simulink model "v2012_PF"  (Simulink 7.6)
(part 2 of 4)

  Line133 : PMComponent  Tag=PSATblock  Description=Power Flow  PhysicalDomain=psatdomain  LeftPortType=p1  RightPortType=p1  LConnTagsString=__newl0  RConnTagsString=__newr0  mask(Line){p3_4_5q=[100  230  60], p6q=9, p8q=[0.023], p9q=[0.00036046], p10q=[0.357e-6], p13_14_15q=[475.8 432.5 475.8], p16q=on}
      mask prompts: p3_4_5q "Power, Voltage and Frequency Ratings [MVA, kV, Hz]"; p6q "Length of line [km] (0 for p.u. parameters)"; p8q "Resistance [p.u. (Ohms/km)]"; p9q "Reactance [p.u. (H/km)]"; p10q "Susceptance [p.u. (F/km)]"; p13_14_15q "Imax, Pmax and Smax [p.u., p.u., p.u.]"; p16q "Connected"
      mask help: This block defines a pi model for a tree phase cable.
      mask init:
      | [x,y] = fm_draw('circle');
      | [x1,y1] = fm_draw('semicircle');
      mask CallbackString: ||||||fm_block
      mask Display:
      | color('yellow')
      | plot(10+0.433*x,0.5+0.433*y)
      | plot(9.567+0.433*x,-0.25+0.433*y)
      | plot(10.433+0.433*x,-0.25+0.433*y)
      | color('black')
      | plot(-x1,y1)
      | plot(10+x,y,[0 10],[1 1],[0 10],[-1 -1])
  Line134 : PMComponent  Tag=PSATblock  Description=Power Flow  PhysicalDomain=psatdomain  LeftPortType=p1  RightPortType=p1  LConnTagsString=__newl0  RConnTagsString=__newr0  mask(Line){p3_4_5q=[100  230  60], p6q=19, p8q=[0.05], p9q=[0.001294461], p10q=[0.008941863e-6], p13_14_15q=[62.8 57.1 62.8], p16q=on}
      mask prompts: p3_4_5q "Power, Voltage and Frequency Ratings [MVA, kV, Hz]"; p6q "Length of line [km] (0 for p.u. parameters)"; p8q "Resistance [p.u. (Ohms/km)]"; p9q "Reactance [p.u. (H/km)]"; p10q "Susceptance [p.u. (F/km)]"; p13_14_15q "Imax, Pmax and Smax [p.u., p.u., p.u.]"; p16q "Connected"
      mask help: This block defines a pi model for a tree phase line.
      mask init:
      | [xp,yp] = fm_draw('pi');
      mask CallbackString: ||||||fm_block
      mask Display:
      | plot([-1  1  1 -1 -1],[-0.2 -0.2 0.2 0.2 -0.2])
      | color('blue')
      | plot(0.35*xp,0.2*yp)
  Line135 : PMComponent  Tag=PSATblock  Description=Power Flow  PhysicalDomain=psatdomain  LeftPortType=p1  RightPortType=p1  LConnTagsString=__newl0  RConnTagsString=__newr0  mask(Line){p3_4_5q=[100  138  60], p6q=15.4, p8q=[0.125], p9q=[0.000994719], p10q=[0.007460394e-6], p13_14_15q=[36.3 33 36.3], p16q=on}
      mask prompts: p3_4_5q "Power, Voltage and Frequency Ratings [MVA, kV, Hz]"; p6q "Length of line [km] (0 for p.u. parameters)"; p8q "Resistance [p.u. (Ohms/km)]"; p9q "Reactance [p.u. (H/km)]"; p10q "Susceptance [p.u. (F/km)]"; p13_14_15q "Imax, Pmax and Smax [p.u., p.u., p.u.]"; p16q "Connected"
      mask help: This block defines a pi model for a tree phase line.
      mask init:
      | [xp,yp] = fm_draw('pi');
      mask CallbackString: ||||||fm_block
      mask Display:
      | plot([-1  1  1 -1 -1],[-0.2 -0.2 0.2 0.2 -0.2])
      | color('blue')
      | plot(0.35*xp,0.2*yp)
  Line136 : PMComponent  Tag=PSATblock  Description=Power Flow  PhysicalDomain=psatdomain  LeftPortType=p1  RightPortType=p1  LConnTagsString=__newl0  RConnTagsString=__newr0  mask(Line){p3_4_5q=[100  138  60], p6q=15.4, p8q=[0.125], p9q=[0.000994719], p10q=[0.007460394e-6], p13_14_15q=[36.3 33 36.3], p16q=on}
      mask prompts: p3_4_5q "Power, Voltage and Frequency Ratings [MVA, kV, Hz]"; p6q "Length of line [km] (0 for p.u. parameters)"; p8q "Resistance [p.u. (Ohms/km)]"; p9q "Reactance [p.u. (H/km)]"; p10q "Susceptance [p.u. (F/km)]"; p13_14_15q "Imax, Pmax and Smax [p.u., p.u., p.u.]"; p16q "Connected"
      mask help: This block defines a pi model for a tree phase line.
      mask init:
      | [xp,yp] = fm_draw('pi');
      mask CallbackString: ||||||fm_block
      mask Display:
      | plot([-1  1  1 -1 -1],[-0.2 -0.2 0.2 0.2 -0.2])
      | color('blue')
      | plot(0.35*xp,0.2*yp)
  Line137 : PMComponent  Tag=PSATblock  Description=Power Flow  PhysicalDomain=psatdomain  LeftPortType=p1  RightPortType=p1  LConnTagsString=__newl0  RConnTagsString=__newr0  mask(Line){p3_4_5q=[100  138  60], p6q=10.7, p8q=[0.125], p9q=[0.000994719], p10q=[0.007460394e-6], p13_14_15q=[52.2 47.5 52.2], p16q=on}
      mask prompts: p3_4_5q "Power, Voltage and Frequency Ratings [MVA, kV, Hz]"; p6q "Length of line [km] (0 for p.u. parameters)"; p8q "Resistance [p.u. (Ohms/km)]"; p9q "Reactance [p.u. (H/km)]"; p10q "Susceptance [p.u. (F/km)]"; p13_14_15q "Imax, Pmax and Smax [p.u., p.u., p.u.]"; p16q "Connected"
      mask help: This block defines a pi model for a tree phase line.
      mask init:
      | [xp,yp] = fm_draw('pi');
      mask CallbackString: ||||||fm_block
      mask Display:
      | plot([-1  1  1 -1 -1],[-0.2 -0.2 0.2 0.2 -0.2])
      | color('blue')
      | plot(0.35*xp,0.2*yp)
  Line138 : PMComponent  Tag=PSATblock  Description=Power Flow  PhysicalDomain=psatdomain  LeftPortType=p1  RightPortType=p1  LConnTagsString=__newl0  RConnTagsString=__newr0  mask(Line){p3_4_5q=[100  230  60], p6q=124, p8q=[0.05], p9q=[0.001294461], p10q=[0.008941863e-6], p13_14_15q=[9.6 8.7 9.6], p16q=on}
      mask prompts: p3_4_5q "Power, Voltage and Frequency Ratings [MVA, kV, Hz]"; p6q "Length of line [km] (0 for p.u. parameters)"; p8q "Resistance [p.u. (Ohms/km)]"; p9q "Reactance [p.u. (H/km)]"; p10q "Susceptance [p.u. (F/km)]"; p13_14_15q "Imax, Pmax and Smax [p.u., p.u., p.u.]"; p16q "Connected"
      mask help: This block defines a pi model for a tree phase line.
      mask init:
      | [xp,yp] = fm_draw('pi');
      mask CallbackString: ||||||fm_block
      mask Display:
      | plot([-1  1  1 -1 -1],[-0.2 -0.2 0.2 0.2 -0.2])
      | color('blue')
      | plot(0.35*xp,0.2*yp)
  Line139 : PMComponent  Tag=PSATblock  Description=Power Flow  PhysicalDomain=psatdomain  LeftPortType=p1  RightPortType=p1  LConnTagsString=__newl0  RConnTagsString=__newr0  mask(Line){p3_4_5q=[100  138  60], p6q=12.2, p8q=[0.125], p9q=[0.000994719], p10q=[0.007460394e-6], p13_14_15q=[45.8 41.6 45.8], p16q=on}
      mask prompts: p3_4_5q "Power, Voltage and Frequency Ratings [MVA, kV, Hz]"; p6q "Length of line [km] (0 for p.u. parameters)"; p8q "Resistance [p.u. (Ohms/km)]"; p9q "Reactance [p.u. (H/km)]"; p10q "Susceptance [p.u. (F/km)]"; p13_14_15q "Imax, Pmax and Smax [p.u., p.u., p.u.]"; p16q "Connected"
      mask help: This block defines a pi model for a tree phase line.
      mask init:
      | [xp,yp] = fm_draw('pi');
      mask CallbackString: ||||||fm_block
      mask Display:
      | plot([-1  1  1 -1 -1],[-0.2 -0.2 0.2 0.2 -0.2])
      | color('blue')
      | plot(0.35*xp,0.2*yp)
  Line14 : PMComponent  Tag=PSATblock  Description=Power Flow  PhysicalDomain=psatdomain  LeftPortType=p1  RightPortType=p1  LConnTagsString=__newl0  RConnTagsString=__newr0  mask(Line){p3_4_5q=[100  230  60], p6q=20.2, p8q=[0.05], p9q=[0.001294461], p10q=[0.008941863e-6], p13_14_15q=[59 53.7 59], p16q=on}
      mask prompts: p3_4_5q "Power, Voltage and Frequency Ratings [MVA, kV, Hz]"; p6q "Length of line [km] (0 for p.u. parameters)"; p8q "Resistance [p.u. (Ohms/km)]"; p9q "Reactance [p.u. (H/km)]"; p10q "Susceptance [p.u. (F/km)]"; p13_14_15q "Imax, Pmax and Smax [p.u., p.u., p.u.]"; p16q "Connected"
      mask help: This block defines a pi model for a tree phase line.
      mask init:
      | [xp,yp] = fm_draw('pi');
      mask CallbackString: ||||||fm_block
      mask Display:
      | plot([-1  1  1 -1 -1],[-0.2 -0.2 0.2 0.2 -0.2])
      | color('blue')
      | plot(0.35*xp,0.2*yp)
  Line140 : PMComponent  Tag=PSATblock  Description=Power Flow  PhysicalDomain=psatdomain  LeftPortType=p1  RightPortType=p1  LConnTagsString=__newl0  RConnTagsString=__newr0  mask(Line){p3_4_5q=[100  765  60], p6q=[65], p8q=[0.012], p9q=[0.0008727], p10q=[0.013204566e-6], p13_14_15q=[25.29 22.76 25.29], p16q=on}
      mask prompts: p3_4_5q "Power, Voltage and Frequency Ratings [MVA, kV, Hz]"; p6q "Length of line [km] (0 for p.u. parameters)"; p8q "Resistance [p.u. (Ohms/km)]"; p9q "Reactance [p.u. (H/km)]"; p10q "Susceptance [p.u. (F/km)]"; p13_14_15q "Imax, Pmax and Smax [p.u., p.u., p.u.]"; p16q "Connected"
      mask help: This block defines a pi model for a tree phase line.
      mask init:
      | [xp,yp] = fm_draw('pi');
      mask CallbackString: ||||||fm_block
      mask Display:
      | plot([-1  1  1 -1 -1],[-0.2 -0.2 0.2 0.2 -0.2])
      | color('blue')
      | plot(0.35*xp,0.2*yp)
  Line141 : PMComponent  Tag=PSATblock  Description=Power Flow  PhysicalDomain=psatdomain  LeftPortType=p1  RightPortType=p1  LConnTagsString=__newl0  RConnTagsString=__newr0  mask(Line){p3_4_5q=[100  230  60], p6q=59, p8q=[0.05], p9q=[0.001294461], p10q=[0.008941863e-6], p13_14_15q=[20.2 18.4 20.2], p16q=on}
      mask prompts: p3_4_5q "Power, Voltage and Frequency Ratings [MVA, kV, Hz]"; p6q "Length of line [km] (0 for p.u. parameters)"; p8q "Resistance [p.u. (Ohms/km)]"; p9q "Reactance [p.u. (H/km)]"; p10q "Susceptance [p.u. (F/km)]"; p13_14_15q "Imax, Pmax and Smax [p.u., p.u., p.u.]"; p16q "Connected"
      mask help: This block defines a pi model for a tree phase line.
      mask init:
      | [xp,yp] = fm_draw('pi');
      mask CallbackString: ||||||fm_block
      mask Display:
      | plot([-1  1  1 -1 -1],[-0.2 -0.2 0.2 0.2 -0.2])
      | color('blue')
      | plot(0.35*xp,0.2*yp)
  Line142 : PMComponent  Tag=PSATblock  Description=Power Flow  PhysicalDomain=psatdomain  LeftPortType=p1  RightPortType=p1  LConnTagsString=__newl0  RConnTagsString=__newr0  mask(Line){p3_4_5q=[100  115  60], p6q=82, p8q=[0.125], p9q=[0.000994719], p10q=[0.007460394e-6], p13_14_15q=[6.8 6.2 6.8], p16q=on}
      mask prompts: p3_4_5q "Power, Voltage and Frequency Ratings [MVA, kV, Hz]"; p6q "Length of line [km] (0 for p.u. parameters)"; p8q "Resistance [p.u. (Ohms/km)]"; p9q "Reactance [p.u. (H/km)]"; p10q "Susceptance [p.u. (F/km)]"; p13_14_15q "Imax, Pmax and Smax [p.u., p.u., p.u.]"; p16q "Connected"
      mask help: This block defines a pi model for a tree phase line.
      mask init:
      | [xp,yp] = fm_draw('pi');
      mask CallbackString: ||||||fm_block
      mask Display:
      | plot([-1  1  1 -1 -1],[-0.2 -0.2 0.2 0.2 -0.2])
      | color('blue')
      | plot(0.35*xp,0.2*yp)
  Line143 : PMComponent  Tag=PSATblock  Description=Power Flow  PhysicalDomain=psatdomain  LeftPortType=p1  RightPortType=p1  LConnTagsString=__newl0  RConnTagsString=__newr0  mask(Line){p3_4_5q=[100  230  60], p6q=111, p8q=[0.05], p9q=[0.001294461], p10q=[0.008941863e-6], p13_14_15q=[10.7 9.8 10.7], p16q=on}
      mask prompts: p3_4_5q "Power, Voltage and Frequency Ratings [MVA, kV, Hz]"; p6q "Length of line [km] (0 for p.u. parameters)"; p8q "Resistance [p.u. (Ohms/km)]"; p9q "Reactance [p.u. (H/km)]"; p10q "Susceptance [p.u. (F/km)]"; p13_14_15q "Imax, Pmax and Smax [p.u., p.u., p.u.]"; p16q "Connected"
      mask help: This block defines a pi model for a tree phase line.
      mask init:
      | [xp,yp] = fm_draw('pi');
      mask CallbackString: ||||||fm_block
      mask Display:
      | plot([-1  1  1 -1 -1],[-0.2 -0.2 0.2 0.2 -0.2])
      | color('blue')
      | plot(0.35*xp,0.2*yp)
  Line144 : PMComponent  Tag=PSATblock  Description=Power Flow  PhysicalDomain=psatdomain  LeftPortType=p1  RightPortType=p1  LConnTagsString=__newl0  RConnTagsString=__newr0  mask(Line){p3_4_5q=[100  400  60], p6q=62.1, p8q=[0.033806452], p9q=[0.000933966], p10q=[0.012626303e-6], p13_14_15q=[80.5 73.2 80.5], p16q=on}
      mask prompts: p3_4_5q "Power, Voltage and Frequency Ratings [MVA, kV, Hz]"; p6q "Length of line [km] (0 for p.u. parameters)"; p8q "Resistance [p.u. (Ohms/km)]"; p9q "Reactance [p.u. (H/km)]"; p10q "Susceptance [p.u. (F/km)]"; p13_14_15q "Imax, Pmax and Smax [p.u., p.u., p.u.]"; p16q "Connected"
      mask help: This block defines a pi model for a tree phase line.
      mask init:
      | [xp,yp] = fm_draw('pi');
      mask CallbackString: ||||||fm_block
      mask Display:
      | plot([-1  1  1 -1 -1],[-0.2 -0.2 0.2 0.2 -0.2])
      | color('blue')
      | plot(0.35*xp,0.2*yp)
  Line145 : PMComponent  Tag=PSATblock  Description=Power Flow  PhysicalDomain=psatdomain  LeftPortType=p1  RightPortType=p1  LConnTagsString=__newl0  RConnTagsString=__newr0  mask(Line){p3_4_5q=[100  115  60], p6q=12, p8q=[0.125], p9q=[0.000994719], p10q=[0.007460394e-6], p13_14_15q=[45.8 41.6 45.8], p16q=on}
      mask prompts: p3_4_5q "Power, Voltage and Frequency Ratings [MVA, kV, Hz]"; p6q "Length of line [km] (0 for p.u. parameters)"; p8q "Resistance [p.u. (Ohms/km)]"; p9q "Reactance [p.u. (H/km)]"; p10q "Susceptance [p.u. (F/km)]"; p13_14_15q "Imax, Pmax and Smax [p.u., p.u., p.u.]"; p16q "Connected"
      mask help: This block defines a pi model for a tree phase line.
      mask init:
      | [xp,yp] = fm_draw('pi');
      mask CallbackString: ||||||fm_block
      mask Display:
      | plot([-1  1  1 -1 -1],[-0.2 -0.2 0.2 0.2 -0.2])
      | color('blue')
      | plot(0.35*xp,0.2*yp)
  Line146 : PMComponent  Tag=PSATblock  Description=Power Flow  PhysicalDomain=psatdomain  LeftPortType=p1  RightPortType=p1  LConnTagsString=__newl0  RConnTagsString=__newr0  mask(Line){p3_4_5q=[100  400  60], p6q=152, p8q=[0.033806452], p9q=[0.000933966], p10q=[0.012626303e-6], p13_14_15q=[32.9 29.9 32.9], p16q=on}
      mask prompts: p3_4_5q "Power, Voltage and Frequency Ratings [MVA, kV, Hz]"; p6q "Length of line [km] (0 for p.u. parameters)"; p8q "Resistance [p.u. (Ohms/km)]"; p9q "Reactance [p.u. (H/km)]"; p10q "Susceptance [p.u. (F/km)]"; p13_14_15q "Imax, Pmax and Smax [p.u., p.u., p.u.]"; p16q "Connected"
      mask help: This block defines a pi model for a tree phase line.
      mask init:
      | [xp,yp] = fm_draw('pi');
      mask CallbackString: ||||||fm_block
      mask Display:
      | plot([-1  1  1 -1 -1],[-0.2 -0.2 0.2 0.2 -0.2])
      | color('blue')
      | plot(0.35*xp,0.2*yp)
  Line147 : PMComponent  Tag=PSATblock  Description=Power Flow  PhysicalDomain=psatdomain  LeftPortType=p1  RightPortType=p1  LConnTagsString=__newl0  RConnTagsString=__newr0  mask(Line){p3_4_5q=[100  400  60], p6q=40, p8q=[0.033806452], p9q=[0.000933966], p10q=[0.012626303e-6], p13_14_15q=[125 114 125], p16q=on}
      mask prompts: p3_4_5q "Power, Voltage and Frequency Ratings [MVA, kV, Hz]"; p6q "Length of line [km] (0 for p.u. parameters)"; p8q "Resistance [p.u. (Ohms/km)]"; p9q "Reactance [p.u. (H/km)]"; p10q "Susceptance [p.u. (F/km)]"; p13_14_15q "Imax, Pmax and Smax [p.u., p.u., p.u.]"; p16q "Connected"
      mask help: This block defines a pi model for a tree phase line.
      mask init:
      | [xp,yp] = fm_draw('pi');
      mask CallbackString: ||||||fm_block
      mask Display:
      | plot([-1  1  1 -1 -1],[-0.2 -0.2 0.2 0.2 -0.2])
      | color('blue')
      | plot(0.35*xp,0.2*yp)
  Line148 : PMComponent  Tag=PSATblock  Description=Power Flow  PhysicalDomain=psatdomain  LeftPortType=p1  RightPortType=p1  LConnTagsString=__newl0  RConnTagsString=__newr0  mask(Line){p3_4_5q=[100  230  60], p6q=197.3, p8q=[0.05], p9q=[0.001294461], p10q=[0.008941863e-6], p13_14_15q=[6 5.5 6], p16q=on}
      mask prompts: p3_4_5q "Power, Voltage and Frequency Ratings [MVA, kV, Hz]"; p6q "Length of line [km] (0 for p.u. parameters)"; p8q "Resistance [p.u. (Ohms/km)]"; p9q "Reactance [p.u. (H/km)]"; p10q "Susceptance [p.u. (F/km)]"; p13_14_15q "Imax, Pmax and Smax [p.u., p.u., p.u.]"; p16q "Connected"
      mask help: This block defines a pi model for a tree phase line.
      mask init:
      | [xp,yp] = fm_draw('pi');
      mask CallbackString: ||||||fm_block
      mask Display:
      | plot([-1  1  1 -1 -1],[-0.2 -0.2 0.2 0.2 -0.2])
      | color('blue')
      | plot(0.35*xp,0.2*yp)
  Line149 : PMComponent  Tag=PSATblock  Description=Power Flow  PhysicalDomain=psatdomain  LeftPortType=p1  RightPortType=p1  LConnTagsString=__newl0  RConnTagsString=__newr0  mask(Line){p3_4_5q=[100  230  60], p6q=206, p8q=[0.05], p9q=[0.001294461], p10q=[0.008941863e-6], p13_14_15q=[5.8 5.3 5.8], p16q=on}
      mask prompts: p3_4_5q "Power, Voltage and Frequency Ratings [MVA, kV, Hz]"; p6q "Length of line [km] (0 for p.u. parameters)"; p8q "Resistance [p.u. (Ohms/km)]"; p9q "Reactance [p.u. (H/km)]"; p10q "Susceptance [p.u. (F/km)]"; p13_14_15q "Imax, Pmax and Smax [p.u., p.u., p.u.]"; p16q "Connected"
      mask help: This block defines a pi model for a tree phase line.
      mask init:
      | [xp,yp] = fm_draw('pi');
      mask CallbackString: ||||||fm_block
      mask Display:
      | plot([-1  1  1 -1 -1],[-0.2 -0.2 0.2 0.2 -0.2])
      | color('blue')
      | plot(0.35*xp,0.2*yp)
  Line15 : PMComponent  Tag=PSATblock  Description=Power Flow  PhysicalDomain=psatdomain  LeftPortType=p1  RightPortType=p1  LConnTagsString=__newl0  RConnTagsString=__newr0  mask(Line){p3_4_5q=[100  400  60], p6q=68, p8q=[0.033806452], p9q=[0.000933966], p10q=[0.012626303e-6], p13_14_15q=[73.5 66.8 73.5], p16q=on}
      mask prompts: p3_4_5q "Power, Voltage and Frequency Ratings [MVA, kV, Hz]"; p6q "Length of line [km] (0 for p.u. parameters)"; p8q "Resistance [p.u. (Ohms/km)]"; p9q "Reactance [p.u. (H/km)]"; p10q "Susceptance [p.u. (F/km)]"; p13_14_15q "Imax, Pmax and Smax [p.u., p.u., p.u.]"; p16q "Connected"
      mask help: This block defines a pi model for a tree phase line.
      mask init:
      | [xp,yp] = fm_draw('pi');
      mask CallbackString: ||||||fm_block
      mask Display:
      | plot([-1  1  1 -1 -1],[-0.2 -0.2 0.2 0.2 -0.2])
      | color('blue')
      | plot(0.35*xp,0.2*yp)
  Line150 : PMComponent  Tag=PSATblock  Description=Power Flow  PhysicalDomain=psatdomain  LeftPortType=p1  RightPortType=p1  LConnTagsString=__newl0  RConnTagsString=__newr0  mask(Line){p3_4_5q=[100  115  60], p6q=10, p8q=[0.125], p9q=[0.000994719], p10q=[0.007460394e-6], p13_14_15q=[45.8 41.6 45.8], p16q=on}
      mask prompts: p3_4_5q "Power, Voltage and Frequency Ratings [MVA, kV, Hz]"; p6q "Length of line [km] (0 for p.u. parameters)"; p8q "Resistance [p.u. (Ohms/km)]"; p9q "Reactance [p.u. (H/km)]"; p10q "Susceptance [p.u. (F/km)]"; p13_14_15q "Imax, Pmax and Smax [p.u., p.u., p.u.]"; p16q "Connected"
      mask help: This block defines a pi model for a tree phase line.
      mask init:
      | [xp,yp] = fm_draw('pi');
      mask CallbackString: ||||||fm_block
      mask Display:
      | plot([-1  1  1 -1 -1],[-0.2 -0.2 0.2 0.2 -0.2])
      | color('blue')
      | plot(0.35*xp,0.2*yp)
  Line151 : PMComponent  Tag=PSATblock  Description=Power Flow  PhysicalDomain=psatdomain  LeftPortType=p1  RightPortType=p1  LConnTagsString=__newl0  RConnTagsString=__newr0  mask(Line){p3_4_5q=[100  230  60], p6q=140, p8q=[0.05], p9q=[0.001294461], p10q=[0.008941863e-6], p13_14_15q=[8.5 7.7 8.5], p16q=on}
      mask prompts: p3_4_5q "Power, Voltage and Frequency Ratings [MVA, kV, Hz]"; p6q "Length of line [km] (0 for p.u. parameters)"; p8q "Resistance [p.u. (Ohms/km)]"; p9q "Reactance [p.u. (H/km)]"; p10q "Susceptance [p.u. (F/km)]"; p13_14_15q "Imax, Pmax and Smax [p.u., p.u., p.u.]"; p16q "Connected"
      mask help: This block defines a pi model for a tree phase line.
      mask init:
      | [xp,yp] = fm_draw('pi');
      mask CallbackString: ||||||fm_block
      mask Display:
      | plot([-1  1  1 -1 -1],[-0.2 -0.2 0.2 0.2 -0.2])
      | color('blue')
      | plot(0.35*xp,0.2*yp)
  Line152 : PMComponent  Tag=PSATblock  Description=Power Flow  PhysicalDomain=psatdomain  LeftPortType=p1  RightPortType=p1  LConnTagsString=__newl0  RConnTagsString=__newr0  mask(Line){p3_4_5q=[100  230  60], p6q=64, p8q=[0.05], p9q=[0.001294461], p10q=[0.008941863e-6], p13_14_15q=[18.6 16.9 18.6], p16q=on}
      mask prompts: p3_4_5q "Power, Voltage and Frequency Ratings [MVA, kV, Hz]"; p6q "Length of line [km] (0 for p.u. parameters)"; p8q "Resistance [p.u. (Ohms/km)]"; p9q "Reactance [p.u. (H/km)]"; p10q "Susceptance [p.u. (F/km)]"; p13_14_15q "Imax, Pmax and Smax [p.u., p.u., p.u.]"; p16q "Connected"
      mask help: This block defines a pi model for a tree phase line.
      mask init:
      | [xp,yp] = fm_draw('pi');
      mask CallbackString: ||||||fm_block
      mask Display:
      | plot([-1  1  1 -1 -1],[-0.2 -0.2 0.2 0.2 -0.2])
      | color('blue')
      | plot(0.35*xp,0.2*yp)
  Line153 : PMComponent  Tag=PSATblock  Description=Power Flow  PhysicalDomain=psatdomain  LeftPortType=p1  RightPortType=p1  LConnTagsString=__newl0  RConnTagsString=__newr0  mask(Line){p3_4_5q=[100  115  60], p6q=10, p8q=[0.125], p9q=[0.000994719], p10q=[0.007460394e-6], p13_14_15q=[45.8 41.6 45.8], p16q=on}
      mask prompts: p3_4_5q "Power, Voltage and Frequency Ratings [MVA, kV, Hz]"; p6q "Length of line [km] (0 for p.u. parameters)"; p8q "Resistance [p.u. (Ohms/km)]"; p9q "Reactance [p.u. (H/km)]"; p10q "Susceptance [p.u. (F/km)]"; p13_14_15q "Imax, Pmax and Smax [p.u., p.u., p.u.]"; p16q "Connected"
      mask help: This block defines a pi model for a tree phase line.
      mask init:
      | [xp,yp] = fm_draw('pi');
      mask CallbackString: ||||||fm_block
      mask Display:
      | plot([-1  1  1 -1 -1],[-0.2 -0.2 0.2 0.2 -0.2])
      | color('blue')
      | plot(0.35*xp,0.2*yp)
  Line154 : PMComponent  Tag=PSATblock  Description=Power Flow  PhysicalDomain=psatdomain  LeftPortType=p1  RightPortType=p1  LConnTagsString=__newl0  RConnTagsString=__newr0  mask(Line){p3_4_5q=[100  115  60], p6q=27, p8q=[0.125], p9q=[0.000994719], p10q=[0.007460394e-6], p13_14_15q=[20.7 18.8 20.7], p16q=on}
      mask prompts: p3_4_5q "Power, Voltage and Frequency Ratings [MVA, kV, Hz]"; p6q "Length of line [km] (0 for p.u. parameters)"; p8q "Resistance [p.u. (Ohms/km)]"; p9q "Reactance [p.u. (H/km)]"; p10q "Susceptance [p.u. (F/km)]"; p13_14_15q "Imax, Pmax and Smax [p.u., p.u., p.u.]"; p16q "Connected"
      mask help: This block defines a pi model for a tree phase line.
      mask init:
      | [xp,yp] = fm_draw('pi');
      mask CallbackString: ||||||fm_block
      mask Display:
      | plot([-1  1  1 -1 -1],[-0.2 -0.2 0.2 0.2 -0.2])
      | color('blue')
      | plot(0.35*xp,0.2*yp)
  Line155 : PMComponent  Tag=PSATblock  Description=Power Flow  PhysicalDomain=psatdomain  LeftPortType=p1  RightPortType=p1  LConnTagsString=__newl0  RConnTagsString=__newr0  mask(Line){p3_4_5q=[100  230  60], p6q=109, p8q=[0.05], p9q=[0.001294461], p10q=[0.008941863e-6], p13_14_15q=[10.9 9.9 10.9], p16q=on}
      mask prompts: p3_4_5q "Power, Voltage and Frequency Ratings [MVA, kV, Hz]"; p6q "Length of line [km] (0 for p.u. parameters)"; p8q "Resistance [p.u. (Ohms/km)]"; p9q "Reactance [p.u. (H/km)]"; p10q "Susceptance [p.u. (F/km)]"; p13_14_15q "Imax, Pmax and Smax [p.u., p.u., p.u.]"; p16q "Connected"
      mask help: This block defines a pi model for a tree phase line.
      mask init:
      | [xp,yp] = fm_draw('pi');
      mask CallbackString: ||||||fm_block
      mask Display:
      | plot([-1  1  1 -1 -1],[-0.2 -0.2 0.2 0.2 -0.2])
      | color('blue')
      | plot(0.35*xp,0.2*yp)
  Line156 : PMComponent  Tag=PSATblock  Description=Power Flow  PhysicalDomain=psatdomain  LeftPortType=p1  RightPortType=p1  LConnTagsString=__newl0  RConnTagsString=__newr0  mask(Line){p3_4_5q=[100  115  60], p6q=29, p8q=[0.023], p9q=[0.00036046], p10q=[0.357e-6], p13_14_15q=[147 134 147], p16q=on}
      mask prompts: p3_4_5q "Power, Voltage and Frequency Ratings [MVA, kV, Hz]"; p6q "Length of line [km] (0 for p.u. parameters)"; p8q "Resistance [p.u. (Ohms/km)]"; p9q "Reactance [p.u. (H/km)]"; p10q "Susceptance [p.u. (F/km)]"; p13_14_15q "Imax, Pmax and Smax [p.u., p.u., p.u.]"; p16q "Connected"
      mask help: This block defines a pi model for a tree phase cable.
      mask init:
      | [x,y] = fm_draw('circle');
      | [x1,y1] = fm_draw('semicircle');
      mask CallbackString: ||||||fm_block
      mask Display:
      | color('yellow')
      | plot(10+0.433*x,0.5+0.433*y)
      | plot(9.567+0.433*x,-0.25+0.433*y)
      | plot(10.433+0.433*x,-0.25+0.433*y)
      | color('black')
      | plot(-x1,y1)
      | plot(10+x,y,[0 10],[1 1],[0 10],[-1 -1])
  Line157 : PMComponent  Tag=PSATblock  Description=Power Flow  PhysicalDomain=psatdomain  LeftPortType=p1  RightPortType=p1  LConnTagsString=__newl0  RConnTagsString=__newr0  mask(Line){p3_4_5q=[100  400  60], p6q=68, p8q=[0.033806452], p9q=[0.000933966], p10q=[0.012626303e-6], p13_14_15q=[73.5 66.8 73.5], p16q=on}
      mask prompts: p3_4_5q "Power, Voltage and Frequency Ratings [MVA, kV, Hz]"; p6q "Length of line [km] (0 for p.u. parameters)"; p8q "Resistance [p.u. (Ohms/km)]"; p9q "Reactance [p.u. (H/km)]"; p10q "Susceptance [p.u. (F/km)]"; p13_14_15q "Imax, Pmax and Smax [p.u., p.u., p.u.]"; p16q "Connected"
      mask help: This block defines a pi model for a tree phase line.
      mask init:
      | [xp,yp] = fm_draw('pi');
      mask CallbackString: ||||||fm_block
      mask Display:
      | plot([-1  1  1 -1 -1],[-0.2 -0.2 0.2 0.2 -0.2])
      | color('blue')
      | plot(0.35*xp,0.2*yp)
  Line158 : PMComponent  Tag=PSATblock  Description=Power Flow  PhysicalDomain=psatdomain  LeftPortType=p1  RightPortType=p1  LConnTagsString=__newl0  RConnTagsString=__newr0  mask(Line){p3_4_5q=[100  230  60], p6q=7, p8q=[0.05], p9q=[0.001294461], p10q=[0.008941863e-6], p13_14_15q=[170 155 170], p16q=on}
      mask prompts: p3_4_5q "Power, Voltage and Frequency Ratings [MVA, kV, Hz]"; p6q "Length of line [km] (0 for p.u. parameters)"; p8q "Resistance [p.u. (Ohms/km)]"; p9q "Reactance [p.u. (H/km)]"; p10q "Susceptance [p.u. (F/km)]"; p13_14_15q "Imax, Pmax and Smax [p.u., p.u., p.u.]"; p16q "Connected"
      mask help: This block defines a pi model for a tree phase line.
      mask init:
      | [xp,yp] = fm_draw('pi');
      mask CallbackString: ||||||fm_block
      mask Display:
      | plot([-1  1  1 -1 -1],[-0.2 -0.2 0.2 0.2 -0.2])
      | color('blue')
      | plot(0.35*xp,0.2*yp)
  Line159 : PMComponent  Tag=PSATblock  Description=Power Flow  PhysicalDomain=psatdomain  LeftPortType=p1  RightPortType=p1  LConnTagsString=__newl0  RConnTagsString=__newr0  mask(Line){p3_4_5q=[100  230  60], p6q=160, p8q=[0.05], p9q=[0.001294461], p10q=[0.008941863e-6], p13_14_15q=[7.5 6.8 7.5], p16q=on}
      mask prompts: p3_4_5q "Power, Voltage and Frequency Ratings [MVA, kV, Hz]"; p6q "Length of line [km] (0 for p.u. parameters)"; p8q "Resistance [p.u. (Ohms/km)]"; p9q "Reactance [p.u. (H/km)]"; p10q "Susceptance [p.u. (F/km)]"; p13_14_15q "Imax, Pmax and Smax [p.u., p.u., p.u.]"; p16q "Connected"
      mask help: This block defines a pi model for a tree phase line.
      mask init:
      | [xp,yp] = fm_draw('pi');
      mask CallbackString: ||||||fm_block
      mask Display:
      | plot([-1  1  1 -1 -1],[-0.2 -0.2 0.2 0.2 -0.2])
      | color('blue')
      | plot(0.35*xp,0.2*yp)
  Line16 : PMComponent  Tag=PSATblock  Description=Power Flow  PhysicalDomain=psatdomain  LeftPortType=p1  RightPortType=p1  LConnTagsString=__newl0  RConnTagsString=__newr0  mask(Line){p3_4_5q=[100  400  60], p6q=132, p8q=[0.033806452], p9q=[0.000933966], p10q=[0.012626303e-6], p13_14_15q=[37.9 34.4 37.9], p16q=on}
      mask prompts: p3_4_5q "Power, Voltage and Frequency Ratings [MVA, kV, Hz]"; p6q "Length of line [km] (0 for p.u. parameters)"; p8q "Resistance [p.u. (Ohms/km)]"; p9q "Reactance [p.u. (H/km)]"; p10q "Susceptance [p.u. (F/km)]"; p13_14_15q "Imax, Pmax and Smax [p.u., p.u., p.u.]"; p16q "Connected"
      mask help: This block defines a pi model for a tree phase line.
      mask init:
      | [xp,yp] = fm_draw('pi');
      mask CallbackString: ||||||fm_block
      mask Display:
      | plot([-1  1  1 -1 -1],[-0.2 -0.2 0.2 0.2 -0.2])
      | color('blue')
      | plot(0.35*xp,0.2*yp)
  Line160 : PMComponent  Tag=PSATblock  Description=Power Flow  PhysicalDomain=psatdomain  LeftPortType=p1  RightPortType=p1  LConnTagsString=__newl0  RConnTagsString=__newr0  mask(Line){p3_4_5q=[100  230  60], p6q=87, p8q=[0.05], p9q=[0.001294461], p10q=[0.008941863e-6], p13_14_15q=[13.7 12.5 13.7], p16q=on}
      mask prompts: p3_4_5q "Power, Voltage and Frequency Ratings [MVA, kV, Hz]"; p6q "Length of line [km] (0 for p.u. parameters)"; p8q "Resistance [p.u. (Ohms/km)]"; p9q "Reactance [p.u. (H/km)]"; p10q "Susceptance [p.u. (F/km)]"; p13_14_15q "Imax, Pmax and Smax [p.u., p.u., p.u.]"; p16q "Connected"
      mask help: This block defines a pi model for a tree phase line.
      mask init:
      | [xp,yp] = fm_draw('pi');
      mask CallbackString: ||||||fm_block
      mask Display:
      | plot([-1  1  1 -1 -1],[-0.2 -0.2 0.2 0.2 -0.2])
      | color('blue')
      | plot(0.35*xp,0.2*yp)
  Line161 : PMComponent  Tag=PSATblock  Description=Power Flow  PhysicalDomain=psatdomain  LeftPortType=p1  RightPortType=p1  LConnTagsString=__newl0  RConnTagsString=__newr0  mask(Line){p3_4_5q=[100  230  60], p6q=2, p8q=[0.05], p9q=[0.001294461], p10q=[0.008941863e-6], p13_14_15q=[596 542 596], p16q=on}
      mask prompts: p3_4_5q "Power, Voltage and Frequency Ratings [MVA, kV, Hz]"; p6q "Length of line [km] (0 for p.u. parameters)"; p8q "Resistance [p.u. (Ohms/km)]"; p9q "Reactance [p.u. (H/km)]"; p10q "Susceptance [p.u. (F/km)]"; p13_14_15q "Imax, Pmax and Smax [p.u., p.u., p.u.]"; p16q "Connected"
      mask help: This block defines a pi model for a tree phase line.
      mask init:
      | [xp,yp] = fm_draw('pi');
      mask CallbackString: ||||||fm_block
      mask Display:
      | plot([-1  1  1 -1 -1],[-0.2 -0.2 0.2 0.2 -0.2])
      | color('blue')
      | plot(0.35*xp,0.2*yp)
  Line162 : PMComponent  Tag=PSATblock  Description=Power Flow  PhysicalDomain=psatdomain  LeftPortType=p1  RightPortType=p1  LConnTagsString=__newl0  RConnTagsString=__newr0  mask(Line){p3_4_5q=[100  115  60], p6q=27, p8q=[0.125], p9q=[0.000994719], p10q=[0.007460394e-6], p13_14_15q=[20.7 18.8 20.7], p16q=on}
      mask prompts: p3_4_5q "Power, Voltage and Frequency Ratings [MVA, kV, Hz]"; p6q "Length of line [km] (0 for p.u. parameters)"; p8q "Resistance [p.u. (Ohms/km)]"; p9q "Reactance [p.u. (H/km)]"; p10q "Susceptance [p.u. (F/km)]"; p13_14_15q "Imax, Pmax and Smax [p.u., p.u., p.u.]"; p16q "Connected"
      mask help: This block defines a pi model for a tree phase line.
      mask init:
      | [xp,yp] = fm_draw('pi');
      mask CallbackString: ||||||fm_block
      mask Display:
      | plot([-1  1  1 -1 -1],[-0.2 -0.2 0.2 0.2 -0.2])
      | color('blue')
      | plot(0.35*xp,0.2*yp)
  Line163 : PMComponent  Tag=PSATblock  Description=Power Flow  PhysicalDomain=psatdomain  LeftPortType=p1  RightPortType=p1  LConnTagsString=__newl0  RConnTagsString=__newr0  mask(Line){p3_4_5q=[100  230  60], p6q=64, p8q=[0.05], p9q=[0.001294461], p10q=[0.008941863e-6], p13_14_15q=[18.6 16.9 18.6], p16q=on}
      mask prompts: p3_4_5q "Power, Voltage and Frequency Ratings [MVA, kV, Hz]"; p6q "Length of line [km] (0 for p.u. parameters)"; p8q "Resistance [p.u. (Ohms/km)]"; p9q "Reactance [p.u. (H/km)]"; p10q "Susceptance [p.u. (F/km)]"; p13_14_15q "Imax, Pmax and Smax [p.u., p.u., p.u.]"; p16q "Connected"
      mask help: This block defines a pi model for a tree phase line.
      mask init:
      | [xp,yp] = fm_draw('pi');
      mask CallbackString: ||||||fm_block
      mask Display:
      | plot([-1  1  1 -1 -1],[-0.2 -0.2 0.2 0.2 -0.2])
      | color('blue')
      | plot(0.35*xp,0.2*yp)
  Line164 : PMComponent  Tag=PSATblock  Description=Power Flow  PhysicalDomain=psatdomain  LeftPortType=p1  RightPortType=p1  LConnTagsString=__newl0  RConnTagsString=__newr0  mask(Line){p3_4_5q=[100  230  60], p6q=30, p8q=[0.05], p9q=[0.001294461], p10q=[0.008941863e-6], p13_14_15q=[39.7 36.1 39.7], p16q=on}
      mask prompts: p3_4_5q "Power, Voltage and Frequency Ratings [MVA, kV, Hz]"; p6q "Length of line [km] (0 for p.u. parameters)"; p8q "Resistance [p.u. (Ohms/km)]"; p9q "Reactance [p.u. (H/km)]"; p10q "Susceptance [p.u. (F/km)]"; p13_14_15q "Imax, Pmax and Smax [p.u., p.u., p.u.]"; p16q "Connected"
      mask help: This block defines a pi model for a tree phase line.
      mask init:
      | [xp,yp] = fm_draw('pi');
      mask CallbackString: ||||||fm_block
      mask Display:
      | plot([-1  1  1 -1 -1],[-0.2 -0.2 0.2 0.2 -0.2])
      | color('blue')
      | plot(0.35*xp,0.2*yp)
  Line165 : PMComponent  Tag=PSATblock  Description=Power Flow  PhysicalDomain=psatdomain  LeftPortType=p1  RightPortType=p1  LConnTagsString=__newl0  RConnTagsString=__newr0  mask(Line){p3_4_5q=[100  115  60], p6q=7, p8q=[0.125], p9q=[0.000994719], p10q=[0.007460394e-6], p13_14_15q=[80 72.5 80], p16q=on}
      mask prompts: p3_4_5q "Power, Voltage and Frequency Ratings [MVA, kV, Hz]"; p6q "Length of line [km] (0 for p.u. parameters)"; p8q "Resistance [p.u. (Ohms/km)]"; p9q "Reactance [p.u. (H/km)]"; p10q "Susceptance [p.u. (F/km)]"; p13_14_15q "Imax, Pmax and Smax [p.u., p.u., p.u.]"; p16q "Connected"
      mask help: This block defines a pi model for a tree phase line.
      mask init:
      | [xp,yp] = fm_draw('pi');
      mask CallbackString: ||||||fm_block
      mask Display:
      | plot([-1  1  1 -1 -1],[-0.2 -0.2 0.2 0.2 -0.2])
      | color('blue')
      | plot(0.35*xp,0.2*yp)
  Line166 : PMComponent  Tag=PSATblock  Description=Power Flow  PhysicalDomain=psatdomain  LeftPortType=p1  RightPortType=p1  LConnTagsString=__newl0  RConnTagsString=__newr0  mask(Line){p3_4_5q=[100  115  60], p6q=7, p8q=[0.125], p9q=[0.000994719], p10q=[0.007460394e-6], p13_14_15q=[80 72.5 80], p16q=on}
      mask prompts: p3_4_5q "Power, Voltage and Frequency Ratings [MVA, kV, Hz]"; p6q "Length of line [km] (0 for p.u. parameters)"; p8q "Resistance [p.u. (Ohms/km)]"; p9q "Reactance [p.u. (H/km)]"; p10q "Susceptance [p.u. (F/km)]"; p13_14_15q "Imax, Pmax and Smax [p.u., p.u., p.u.]"; p16q "Connected"
      mask help: This block defines a pi model for a tree phase line.
      mask init:
      | [xp,yp] = fm_draw('pi');
      mask CallbackString: ||||||fm_block
      mask Display:
      | plot([-1  1  1 -1 -1],[-0.2 -0.2 0.2 0.2 -0.2])
      | color('blue')
      | plot(0.35*xp,0.2*yp)
  Line167 : PMComponent  Tag=PSATblock  Description=Power Flow  PhysicalDomain=psatdomain  LeftPortType=p1  RightPortType=p1  LConnTagsString=__newl0  RConnTagsString=__newr0  mask(Line){p3_4_5q=[100  115  60], p6q=7, p8q=[0.125], p9q=[0.000994719], p10q=[0.007460394e-6], p13_14_15q=[80 72.5 80], p16q=on}
      mask prompts: p3_4_5q "Power, Voltage and Frequency Ratings [MVA, kV, Hz]"; p6q "Length of line [km] (0 for p.u. parameters)"; p8q "Resistance [p.u. (Ohms/km)]"; p9q "Reactance [p.u. (H/km)]"; p10q "Susceptance [p.u. (F/km)]"; p13_14_15q "Imax, Pmax and Smax [p.u., p.u., p.u.]"; p16q "Connected"
      mask help: This block defines a pi model for a tree phase line.
      mask init:
      | [xp,yp] = fm_draw('pi');
      mask CallbackString: ||||||fm_block
      mask Display:
      | plot([-1  1  1 -1 -1],[-0.2 -0.2 0.2 0.2 -0.2])
      | color('blue')
      | plot(0.35*xp,0.2*yp)
  Line168 : PMComponent  Tag=PSATblock  Description=Power Flow  PhysicalDomain=psatdomain  LeftPortType=p1  RightPortType=p1  LConnTagsString=__newl0  RConnTagsString=__newr0  mask(Line){p3_4_5q=[100  115  60], p6q=7, p8q=[0.125], p9q=[0.000994719], p10q=[0.007460394e-6], p13_14_15q=[80 72.5 80], p16q=on}
      mask prompts: p3_4_5q "Power, Voltage and Frequency Ratings [MVA, kV, Hz]"; p6q "Length of line [km] (0 for p.u. parameters)"; p8q "Resistance [p.u. (Ohms/km)]"; p9q "Reactance [p.u. (H/km)]"; p10q "Susceptance [p.u. (F/km)]"; p13_14_15q "Imax, Pmax and Smax [p.u., p.u., p.u.]"; p16q "Connected"
      mask help: This block defines a pi model for a tree phase line.
      mask init:
      | [xp,yp] = fm_draw('pi');
      mask CallbackString: ||||||fm_block
      mask Display:
      | plot([-1  1  1 -1 -1],[-0.2 -0.2 0.2 0.2 -0.2])
      | color('blue')
      | plot(0.35*xp,0.2*yp)
  Line169 : PMComponent  Tag=PSATblock  Description=Power Flow  PhysicalDomain=psatdomain  LeftPortType=p1  RightPortType=p1  LConnTagsString=__newl0  RConnTagsString=__newr0  mask(Line){p3_4_5q=[100  115  60], p6q=68, p8q=[0.125], p9q=[0.000994719], p10q=[0.007460394e-6], p13_14_15q=[8.2 7.5 8.2], p16q=on}
      mask prompts: p3_4_5q "Power, Voltage and Frequency Ratings [MVA, kV, Hz]"; p6q "Length of line [km] (0 for p.u. parameters)"; p8q "Resistance [p.u. (Ohms/km)]"; p9q "Reactance [p.u. (H/km)]"; p10q "Susceptance [p.u. (F/km)]"; p13_14_15q "Imax, Pmax and Smax [p.u., p.u., p.u.]"; p16q "Connected"
      mask help: This block defines a pi model for a tree phase line.
      mask init:
      | [xp,yp] = fm_draw('pi');
      mask CallbackString: ||||||fm_block
      mask Display:
      | plot([-1  1  1 -1 -1],[-0.2 -0.2 0.2 0.2 -0.2])
      | color('blue')
      | plot(0.35*xp,0.2*yp)
  Line17 : PMComponent  Tag=PSATblock  Description=Power Flow  PhysicalDomain=psatdomain  LeftPortType=p1  RightPortType=p1  LConnTagsString=__newl0  RConnTagsString=__newr0  mask(Line){p3_4_5q=[100  400  60], p6q=56, p8q=[0.033806452], p9q=[0.000933966], p10q=[0.012626303e-6], p13_14_15q=[89.3 81.1 89.3], p16q=on}
      mask prompts: p3_4_5q "Power, Voltage and Frequency Ratings [MVA, kV, Hz]"; p6q "Length of line [km] (0 for p.u. parameters)"; p8q "Resistance [p.u. (Ohms/km)]"; p9q "Reactance [p.u. (H/km)]"; p10q "Susceptance [p.u. (F/km)]"; p13_14_15q "Imax, Pmax and Smax [p.u., p.u., p.u.]"; p16q "Connected"
      mask help: This block defines a pi model for a tree phase line.
      mask init:
      | [xp,yp] = fm_draw('pi');
      mask CallbackString: ||||||fm_block
      mask Display:
      | plot([-1  1  1 -1 -1],[-0.2 -0.2 0.2 0.2 -0.2])
      | color('blue')
      | plot(0.35*xp,0.2*yp)
  Line170 : PMComponent  Tag=PSATblock  Description=Power Flow  PhysicalDomain=psatdomain  LeftPortType=p1  RightPortType=p1  LConnTagsString=__newl0  RConnTagsString=__newr0  mask(Line){p3_4_5q=[100  115  60], p6q=71, p8q=[0.125], p9q=[0.000994719], p10q=[0.007460394e-6], p13_14_15q=[8.2 7.5 8.2], p16q=on}
      mask prompts: p3_4_5q "Power, Voltage and Frequency Ratings [MVA, kV, Hz]"; p6q "Length of line [km] (0 for p.u. parameters)"; p8q "Resistance [p.u. (Ohms/km)]"; p9q "Reactance [p.u. (H/km)]"; p10q "Susceptance [p.u. (F/km)]"; p13_14_15q "Imax, Pmax and Smax [p.u., p.u., p.u.]"; p16q "Connected"
      mask help: This block defines a pi model for a tree phase line.
      mask init:
      | [xp,yp] = fm_draw('pi');
      mask CallbackString: ||||||fm_block
      mask Display:
      | plot([-1  1  1 -1 -1],[-0.2 -0.2 0.2 0.2 -0.2])
      | color('blue')
      | plot(0.35*xp,0.2*yp)
  Line171 : PMComponent  Tag=PSATblock  Description=Power Flow  PhysicalDomain=psatdomain  LeftPortType=p1  RightPortType=p1  LConnTagsString=__newl0  RConnTagsString=__newr0  mask(Line){p3_4_5q=[100  115  60], p6q=51, p8q=[0.125], p9q=[0.000994719], p10q=[0.007460394e-6], p13_14_15q=[11 10 11], p16q=on}
      mask prompts: p3_4_5q "Power, Voltage and Frequency Ratings [MVA, kV, Hz]"; p6q "Length of line [km] (0 for p.u. parameters)"; p8q "Resistance [p.u. (Ohms/km)]"; p9q "Reactance [p.u. (H/km)]"; p10q "Susceptance [p.u. (F/km)]"; p13_14_15q "Imax, Pmax and Smax [p.u., p.u., p.u.]"; p16q "Connected"
      mask help: This block defines a pi model for a tree phase line.
      mask init:
      | [xp,yp] = fm_draw('pi');
      mask CallbackString: ||||||fm_block
      mask Display:
      | plot([-1  1  1 -1 -1],[-0.2 -0.2 0.2 0.2 -0.2])
      | color('blue')
      | plot(0.35*xp,0.2*yp)
  Line172 : PMComponent  Tag=PSATblock  Description=Power Flow  PhysicalDomain=psatdomain  LeftPortType=p1  RightPortType=p1  LConnTagsString=__newl0  RConnTagsString=__newr0  mask(Line){p3_4_5q=[100  115  60], p6q=51, p8q=[0.125], p9q=[0.000994719], p10q=[0.007460394e-6], p13_14_15q=[11 10 11], p16q=on}
      mask prompts: p3_4_5q "Power, Voltage and Frequency Ratings [MVA, kV, Hz]"; p6q "Length of line [km] (0 for p.u. parameters)"; p8q "Resistance [p.u. (Ohms/km)]"; p9q "Reactance [p.u. (H/km)]"; p10q "Susceptance [p.u. (F/km)]"; p13_14_15q "Imax, Pmax and Smax [p.u., p.u., p.u.]"; p16q "Connected"
      mask help: This block defines a pi model for a tree phase line.
      mask init:
      | [xp,yp] = fm_draw('pi');
      mask CallbackString: ||||||fm_block
      mask Display:
      | plot([-1  1  1 -1 -1],[-0.2 -0.2 0.2 0.2 -0.2])
      | color('blue')
      | plot(0.35*xp,0.2*yp)
  Line173 : PMComponent  Tag=PSATblock  Description=Power Flow  PhysicalDomain=psatdomain  LeftPortType=p1  RightPortType=p1  LConnTagsString=__newl0  RConnTagsString=__newr0  mask(Line){p3_4_5q=[100  115  60], p6q=82, p8q=[0.125], p9q=[0.000994719], p10q=[0.007460394e-6], p13_14_15q=[6.8 6.2 6.8], p16q=on}
      mask prompts: p3_4_5q "Power, Voltage and Frequency Ratings [MVA, kV, Hz]"; p6q "Length of line [km] (0 for p.u. parameters)"; p8q "Resistance [p.u. (Ohms/km)]"; p9q "Reactance [p.u. (H/km)]"; p10q "Susceptance [p.u. (F/km)]"; p13_14_15q "Imax, Pmax and Smax [p.u., p.u., p.u.]"; p16q "Connected"
      mask help: This block defines a pi model for a tree phase line.
      mask init:
      | [xp,yp] = fm_draw('pi');
      mask CallbackString: ||||||fm_block
      mask Display:
      | plot([-1  1  1 -1 -1],[-0.2 -0.2 0.2 0.2 -0.2])
      | color('blue')
      | plot(0.35*xp,0.2*yp)
  Line174 : PMComponent  Tag=PSATblock  Description=Power Flow  PhysicalDomain=psatdomain  LeftPortType=p1  RightPortType=p1  LConnTagsString=__newl0  RConnTagsString=__newr0  mask(Line){p3_4_5q=[100  230  60], p6q=150, p8q=[0.05], p9q=[0.001294461], p10q=[0.008941863e-6], p13_14_15q=[7.9 7.2 7.9], p16q=on}
      mask prompts: p3_4_5q "Power, Voltage and Frequency Ratings [MVA, kV, Hz]"; p6q "Length of line [km] (0 for p.u. parameters)"; p8q "Resistance [p.u. (Ohms/km)]"; p9q "Reactance [p.u. (H/km)]"; p10q "Susceptance [p.u. (F/km)]"; p13_14_15q "Imax, Pmax and Smax [p.u., p.u., p.u.]"; p16q "Connected"
      mask help: This block defines a pi model for a tree phase line.
      mask init:
      | [xp,yp] = fm_draw('pi');
      mask CallbackString: ||||||fm_block
      mask Display:
      | plot([-1  1  1 -1 -1],[-0.2 -0.2 0.2 0.2 -0.2])
      | color('blue')
      | plot(0.35*xp,0.2*yp)
  Line175 : PMComponent  Tag=PSATblock  Description=Power Flow  PhysicalDomain=psatdomain  LeftPortType=p1  RightPortType=p1  LConnTagsString=__newl0  RConnTagsString=__newr0  mask(Line){p3_4_5q=[100  230  60], p6q=13, p8q=[0.05], p9q=[0.001294461], p10q=[0.008941863e-6], p13_14_15q=[91.7 83.4 91.7], p16q=on}
      mask prompts: p3_4_5q "Power, Voltage and Frequency Ratings [MVA, kV, Hz]"; p6q "Length of line [km] (0 for p.u. parameters)"; p8q "Resistance [p.u. (Ohms/km)]"; p9q "Reactance [p.u. (H/km)]"; p10q "Susceptance [p.u. (F/km)]"; p13_14_15q "Imax, Pmax and Smax [p.u., p.u., p.u.]"; p16q "Connected"
      mask help: This block defines a pi model for a tree phase line.
      mask init:
      | [xp,yp] = fm_draw('pi');
      mask CallbackString: ||||||fm_block
      mask Display:
      | plot([-1  1  1 -1 -1],[-0.2 -0.2 0.2 0.2 -0.2])
      | color('blue')
      | plot(0.35*xp,0.2*yp)
  Line176 : PMComponent  Tag=PSATblock  Description=Power Flow  PhysicalDomain=psatdomain  LeftPortType=p1  RightPortType=p1  LConnTagsString=__newl0  RConnTagsString=__newr0  mask(Line){p3_4_5q=[100  230  60], p6q=44, p8q=[0.05], p9q=[0.001294461], p10q=[0.008941863e-6], p13_14_15q=[27.1 24.6 27.1], p16q=on}
      mask prompts: p3_4_5q "Power, Voltage and Frequency Ratings [MVA, kV, Hz]"; p6q "Length of line [km] (0 for p.u. parameters)"; p8q "Resistance [p.u. (Ohms/km)]"; p9q "Reactance [p.u. (H/km)]"; p10q "Susceptance [p.u. (F/km)]"; p13_14_15q "Imax, Pmax and Smax [p.u., p.u., p.u.]"; p16q "Connected"
      mask help: This block defines a pi model for a tree phase line.
      mask init:
      | [xp,yp] = fm_draw('pi');
      mask CallbackString: ||||||fm_block
      mask Display:
      | plot([-1  1  1 -1 -1],[-0.2 -0.2 0.2 0.2 -0.2])
      | color('blue')
      | plot(0.35*xp,0.2*yp)
  Line177 : PMComponent  Tag=PSATblock  Description=Power Flow  PhysicalDomain=psatdomain  LeftPortType=p1  RightPortType=p1  LConnTagsString=__newl0  RConnTagsString=__newr0  mask(Line){p3_4_5q=[100  230  60], p6q=133, p8q=[0.05], p9q=[0.001294461], p10q=[0.008941863e-6], p13_14_15q=[9 8.2 9], p16q=on}
      mask prompts: p3_4_5q "Power, Voltage and Frequency Ratings [MVA, kV, Hz]"; p6q "Length of line [km] (0 for p.u. parameters)"; p8q "Resistance [p.u. (Ohms/km)]"; p9q "Reactance [p.u. (H/km)]"; p10q "Susceptance [p.u. (F/km)]"; p13_14_15q "Imax, Pmax and Smax [p.u., p.u., p.u.]"; p16q "Connected"
      mask help: This block defines a pi model for a tree phase line.
      mask init:
      | [xp,yp] = fm_draw('pi');
      mask CallbackString: ||||||fm_block
      mask Display:
      | plot([-1  1  1 -1 -1],[-0.2 -0.2 0.2 0.2 -0.2])
      | color('blue')
      | plot(0.35*xp,0.2*yp)
  Line178 : PMComponent  Tag=PSATblock  Description=Power Flow  PhysicalDomain=psatdomain  LeftPortType=p1  RightPortType=p1  LConnTagsString=__newl0  RConnTagsString=__newr0  mask(Line){p3_4_5q=[100  230  60], p6q=10, p8q=[0.05], p9q=[0.001294461], p10q=[0.008941863e-6], p13_14_15q=[119 108 119], p16q=on}
      mask prompts: p3_4_5q "Power, Voltage and Frequency Ratings [MVA, kV, Hz]"; p6q "Length of line [km] (0 for p.u. parameters)"; p8q "Resistance [p.u. (Ohms/km)]"; p9q "Reactance [p.u. (H/km)]"; p10q "Susceptance [p.u. (F/km)]"; p13_14_15q "Imax, Pmax and Smax [p.u., p.u., p.u.]"; p16q "Connected"
      mask help: This block defines a pi model for a tree phase line.
      mask init:
      | [xp,yp] = fm_draw('pi');
      mask CallbackString: ||||||fm_block
      mask Display:
      | plot([-1  1  1 -1 -1],[-0.2 -0.2 0.2 0.2 -0.2])
      | color('blue')
      | plot(0.35*xp,0.2*yp)
  Line179 : PMComponent  Tag=PSATblock  Description=Power Flow  PhysicalDomain=psatdomain  LeftPortType=p1  RightPortType=p1  LConnTagsString=__newl0  RConnTagsString=__newr0  mask(Line){p3_4_5q=[100  230  60], p6q=10, p8q=[0.05], p9q=[0.001294461], p10q=[0.008941863e-6], p13_14_15q=[119 108 119], p16q=on}
      mask prompts: p3_4_5q "Power, Voltage and Frequency Ratings [MVA, kV, Hz]"; p6q "Length of line [km] (0 for p.u. parameters)"; p8q "Resistance [p.u. (Ohms/km)]"; p9q "Reactance [p.u. (H/km)]"; p10q "Susceptance [p.u. (F/km)]"; p13_14_15q "Imax, Pmax and Smax [p.u., p.u., p.u.]"; p16q "Connected"
      mask help: This block defines a pi model for a tree phase line.
      mask init:
      | [xp,yp] = fm_draw('pi');
      mask CallbackString: ||||||fm_block
      mask Display:
      | plot([-1  1  1 -1 -1],[-0.2 -0.2 0.2 0.2 -0.2])
      | color('blue')
      | plot(0.35*xp,0.2*yp)
  Line18 : PMComponent  Tag=PSATblock  Description=Power Flow  PhysicalDomain=psatdomain  LeftPortType=p1  RightPortType=p1  LConnTagsString=__newl0  RConnTagsString=__newr0  mask(Line){p3_4_5q=[100  400  60], p6q=187, p8q=[0.033806452], p9q=[0.000933966], p10q=[0.012626303e-6], p13_14_15q=[26.7 24.3 26.7], p16q=on}
      mask prompts: p3_4_5q "Power, Voltage and Frequency Ratings [MVA, kV, Hz]"; p6q "Length of line [km] (0 for p.u. parameters)"; p8q "Resistance [p.u. (Ohms/km)]"; p9q "Reactance [p.u. (H/km)]"; p10q "Susceptance [p.u. (F/km)]"; p13_14_15q "Imax, Pmax and Smax [p.u., p.u., p.u.]"; p16q "Connected"
      mask help: This block defines a pi model for a tree phase line.
      mask init:
      | [xp,yp] = fm_draw('pi');
      mask CallbackString: ||||||fm_block
      mask Display:
      | plot([-1  1  1 -1 -1],[-0.2 -0.2 0.2 0.2 -0.2])
      | color('blue')
      | plot(0.35*xp,0.2*yp)
  Line182 : PMComponent  Tag=PSATblock  Description=Power Flow  PhysicalDomain=psatdomain  LeftPortType=p1  RightPortType=p1  LConnTagsString=__newl0  RConnTagsString=__newr0  mask(Line){p3_4_5q=[100  400  60], p6q=10, p8q=[0.033806452], p9q=[0.000933966], p10q=[0.012626303e-6], p13_14_15q=[500 454 500], p16q=on}
      mask prompts: p3_4_5q "Power, Voltage and Frequency Ratings [MVA, kV, Hz]"; p6q "Length of line [km] (0 for p.u. parameters)"; p8q "Resistance [p.u. (Ohms/km)]"; p9q "Reactance [p.u. (H/km)]"; p10q "Susceptance [p.u. (F/km)]"; p13_14_15q "Imax, Pmax and Smax [p.u., p.u., p.u.]"; p16q "Connected"
      mask help: This block defines a pi model for a tree phase line.
      mask init:
      | [xp,yp] = fm_draw('pi');
      mask CallbackString: ||||||fm_block
      mask Display:
      | plot([-1  1  1 -1 -1],[-0.2 -0.2 0.2 0.2 -0.2])
      | color('blue')
      | plot(0.35*xp,0.2*yp)
  Line183 : PMComponent  Tag=PSATblock  Description=Power Flow  PhysicalDomain=psatdomain  LeftPortType=p1  RightPortType=p1  LConnTagsString=__newl0  RConnTagsString=__newr0  mask(Line){p3_4_5q=[100  400  60], p6q=10, p8q=[0.033806452], p9q=[0.000933966], p10q=[0.012626303e-6], p13_14_15q=[500 454 500], p16q=on}
      mask prompts: p3_4_5q "Power, Voltage and Frequency Ratings [MVA, kV, Hz]"; p6q "Length of line [km] (0 for p.u. parameters)"; p8q "Resistance [p.u. (Ohms/km)]"; p9q "Reactance [p.u. (H/km)]"; p10q "Susceptance [p.u. (F/km)]"; p13_14_15q "Imax, Pmax and Smax [p.u., p.u., p.u.]"; p16q "Connected"
      mask help: This block defines a pi model for a tree phase line.
      mask init:
      | [xp,yp] = fm_draw('pi');
      mask CallbackString: ||||||fm_block
      mask Display:
      | plot([-1  1  1 -1 -1],[-0.2 -0.2 0.2 0.2 -0.2])
      | color('blue')
      | plot(0.35*xp,0.2*yp)
  Line186 : PMComponent  Tag=PSATblock  Description=Power Flow  PhysicalDomain=psatdomain  LeftPortType=p1  RightPortType=p1  LConnTagsString=__newl0  RConnTagsString=__newr0  mask(Line){p3_4_5q=[100  115  60], p6q=29.67, p8q=[0.125], p9q=[0.000994719], p10q=[0.007460394e-6], p13_14_15q=[0.0 0.0 0.0], p16q=on}
      mask prompts: p3_4_5q "Power, Voltage and Frequency Ratings [MVA, kV, Hz]"; p6q "Length of line [km] (0 for p.u. parameters)"; p8q "Resistance [p.u. (Ohms/km)]"; p9q "Reactance [p.u. (H/km)]"; p10q "Susceptance [p.u. (F/km)]"; p13_14_15q "Imax, Pmax and Smax [p.u., p.u., p.u.]"; p16q "Connected"
      mask help: This block defines a pi model for a tree phase line.
      mask init:
      | [xp,yp] = fm_draw('pi');
      mask CallbackString: ||||||fm_block
      mask Display:
      | plot([-1  1  1 -1 -1],[-0.2 -0.2 0.2 0.2 -0.2])
      | color('blue')
      | plot(0.35*xp,0.2*yp)
  Line187 : PMComponent  Tag=PSATblock  Description=Power Flow  PhysicalDomain=psatdomain  LeftPortType=p1  RightPortType=p1  LConnTagsString=__newl0  RConnTagsString=__newr0  mask(Line){p3_4_5q=[100  115  60], p6q=29.67, p8q=[0.125], p9q=[0.000994719], p10q=[0.007460394e-6], p13_14_15q=[0.0 0.0 0.0], p16q=on}
      mask prompts: p3_4_5q "Power, Voltage and Frequency Ratings [MVA, kV, Hz]"; p6q "Length of line [km] (0 for p.u. parameters)"; p8q "Resistance [p.u. (Ohms/km)]"; p9q "Reactance [p.u. (H/km)]"; p10q "Susceptance [p.u. (F/km)]"; p13_14_15q "Imax, Pmax and Smax [p.u., p.u., p.u.]"; p16q "Connected"
      mask help: This block defines a pi model for a tree phase line.
      mask init:
      | [xp,yp] = fm_draw('pi');
      mask CallbackString: ||||||fm_block
      mask Display:
      | plot([-1  1  1 -1 -1],[-0.2 -0.2 0.2 0.2 -0.2])
      | color('blue')
      | plot(0.35*xp,0.2*yp)
  Line188 : PMComponent  Tag=PSATblock  Description=Power Flow  PhysicalDomain=psatdomain  LeftPortType=p1  RightPortType=p1  LConnTagsString=__newl0  RConnTagsString=__newr0  mask(Line){p3_4_5q=[100  115  60], p6q=14.35, p8q=[0.125], p9q=[0.000994719], p10q=[0.007460394e-6], p13_14_15q=[0.0 0.0 0.0], p16q=on}
      mask prompts: p3_4_5q "Power, Voltage and Frequency Ratings [MVA, kV, Hz]"; p6q "Length of line [km] (0 for p.u. parameters)"; p8q "Resistance [p.u. (Ohms/km)]"; p9q "Reactance [p.u. (H/km)]"; p10q "Susceptance [p.u. (F/km)]"; p13_14_15q "Imax, Pmax and Smax [p.u., p.u., p.u.]"; p16q "Connected"
      mask help: This block defines a pi model for a tree phase line.
      mask init:
      | [xp,yp] = fm_draw('pi');
      mask CallbackString: ||||||fm_block
      mask Display:
      | plot([-1  1  1 -1 -1],[-0.2 -0.2 0.2 0.2 -0.2])
      | color('blue')
      | plot(0.35*xp,0.2*yp)
  Line189 : PMComponent  Tag=PSATblock  Description=Power Flow  PhysicalDomain=psatdomain  LeftPortType=p1  RightPortType=p1  LConnTagsString=__newl0  RConnTagsString=__newr0  mask(Line){p3_4_5q=[100  115  60], p6q=11.47, p8q=[0.125], p9q=[0.000994719], p10q=[0.007460394e-6], p13_14_15q=[0.0 0.0 0.0], p16q=on}
      mask prompts: p3_4_5q "Power, Voltage and Frequency Ratings [MVA, kV, Hz]"; p6q "Length of line [km] (0 for p.u. parameters)"; p8q "Resistance [p.u. (Ohms/km)]"; p9q "Reactance [p.u. (H/km)]"; p10q "Susceptance [p.u. (F/km)]"; p13_14_15q "Imax, Pmax and Smax [p.u., p.u., p.u.]"; p16q "Connected"
      mask help: This block defines a pi model for a tree phase line.
      mask init:
      | [xp,yp] = fm_draw('pi');
      mask CallbackString: ||||||fm_block
      mask Display:
      | plot([-1  1  1 -1 -1],[-0.2 -0.2 0.2 0.2 -0.2])
      | color('blue')
      | plot(0.35*xp,0.2*yp)
  Line19 : PMComponent  Tag=PSATblock  Description=Power Flow  PhysicalDomain=psatdomain  LeftPortType=p1  RightPortType=p1  LConnTagsString=__newl0  RConnTagsString=__newr0  mask(Line){p3_4_5q=[100  230  60], p6q=68, p8q=[0.05], p9q=[0.001294461], p10q=[0.008941863e-6], p13_14_15q=[17.5 15.9 17.5], p16q=on}
      mask prompts: p3_4_5q "Power, Voltage and Frequency Ratings [MVA, kV, Hz]"; p6q "Length of line [km] (0 for p.u. parameters)"; p8q "Resistance [p.u. (Ohms/km)]"; p9q "Reactance [p.u. (H/km)]"; p10q "Susceptance [p.u. (F/km)]"; p13_14_15q "Imax, Pmax and Smax [p.u., p.u., p.u.]"; p16q "Connected"
      mask help: This block defines a pi model for a tree phase line.
      mask init:
      | [xp,yp] = fm_draw('pi');
      mask CallbackString: ||||||fm_block
      mask Display:
      | plot([-1  1  1 -1 -1],[-0.2 -0.2 0.2 0.2 -0.2])
      | color('blue')
      | plot(0.35*xp,0.2*yp)
  Line190 : PMComponent  Tag=PSATblock  Description=Power Flow  PhysicalDomain=psatdomain  LeftPortType=p1  RightPortType=p1  LConnTagsString=__newl0  RConnTagsString=__newr0  mask(Line){p3_4_5q=[100  115  60], p6q=34.72, p8q=[0.125], p9q=[0.000994719], p10q=[0.007460394e-6], p13_14_15q=[0.0 0.0 0.0], p16q=on}
      mask prompts: p3_4_5q "Power, Voltage and Frequency Ratings [MVA, kV, Hz]"; p6q "Length of line [km] (0 for p.u. parameters)"; p8q "Resistance [p.u. (Ohms/km)]"; p9q "Reactance [p.u. (H/km)]"; p10q "Susceptance [p.u. (F/km)]"; p13_14_15q "Imax, Pmax and Smax [p.u., p.u., p.u.]"; p16q "Connected"
      mask help: This block defines a pi model for a tree phase line.
      mask init:
      | [xp,yp] = fm_draw('pi');
      mask CallbackString: ||||||fm_block
      mask Display:
      | plot([-1  1  1 -1 -1],[-0.2 -0.2 0.2 0.2 -0.2])
      | color('blue')
      | plot(0.35*xp,0.2*yp)
  Line191 : PMComponent  Tag=PSATblock  Description=Power Flow  PhysicalDomain=psatdomain  LeftPortType=p1  RightPortType=p1  LConnTagsString=__newl0  RConnTagsString=__newr0  mask(Line){p3_4_5q=[100  115  60], p6q=24.00, p8q=[0.125], p9q=[0.000994719], p10q=[0.007460394e-6], p13_14_15q=[0.0 0.0 0.0], p16q=on}
      mask prompts: p3_4_5q "Power, Voltage and Frequency Ratings [MVA, kV, Hz]"; p6q "Length of line [km] (0 for p.u. parameters)"; p8q "Resistance [p.u. (Ohms/km)]"; p9q "Reactance [p.u. (H/km)]"; p10q "Susceptance [p.u. (F/km)]"; p13_14_15q "Imax, Pmax and Smax [p.u., p.u., p.u.]"; p16q "Connected"
      mask help: This block defines a pi model for a tree phase line.
      mask init:
      | [xp,yp] = fm_draw('pi');
      mask CallbackString: ||||||fm_block
      mask Display:
      | plot([-1  1  1 -1 -1],[-0.2 -0.2 0.2 0.2 -0.2])
      | color('blue')
      | plot(0.35*xp,0.2*yp)
  Line192 : PMComponent  Tag=PSATblock  Description=Power Flow  PhysicalDomain=psatdomain  LeftPortType=p1  RightPortType=p1  LConnTagsString=__newl0  RConnTagsString=__newr0  mask(Line){p3_4_5q=[100  115  60], p6q=6.33, p8q=[0.125], p9q=[0.000994719], p10q=[0.007460394e-6], p13_14_15q=[0.0 0.0 0.0], p16q=on}
      mask prompts: p3_4_5q "Power, Voltage and Frequency Ratings [MVA, kV, Hz]"; p6q "Length of line [km] (0 for p.u. parameters)"; p8q "Resistance [p.u. (Ohms/km)]"; p9q "Reactance [p.u. (H/km)]"; p10q "Susceptance [p.u. (F/km)]"; p13_14_15q "Imax, Pmax and Smax [p.u., p.u., p.u.]"; p16q "Connected"
      mask help: This block defines a pi model for a tree phase line.
      mask init:
      | [xp,yp] = fm_draw('pi');
      mask CallbackString: ||||||fm_block
      mask Display:
      | plot([-1  1  1 -1 -1],[-0.2 -0.2 0.2 0.2 -0.2])
      | color('blue')
      | plot(0.35*xp,0.2*yp)
  Line193 : PMComponent  Tag=PSATblock  Description=Power Flow  PhysicalDomain=psatdomain  LeftPortType=p1  RightPortType=p1  LConnTagsString=__newl0  RConnTagsString=__newr0  mask(Line){p3_4_5q=[100  115  60], p6q=111.46, p8q=[0.125], p9q=[0.000994719], p10q=[0.007460394e-6], p13_14_15q=[0.0 0.0 0.0], p16q=on}
      mask prompts: p3_4_5q "Power, Voltage and Frequency Ratings [MVA, kV, Hz]"; p6q "Length of line [km] (0 for p.u. parameters)"; p8q "Resistance [p.u. (Ohms/km)]"; p9q "Reactance [p.u. (H/km)]"; p10q "Susceptance [p.u. (F/km)]"; p13_14_15q "Imax, Pmax and Smax [p.u., p.u., p.u.]"; p16q "Connected"
      mask help: This block defines a pi model for a tree phase line.
      mask init:
      | [xp,yp] = fm_draw('pi');
      mask CallbackString: ||||||fm_block
      mask Display:
      | plot([-1  1  1 -1 -1],[-0.2 -0.2 0.2 0.2 -0.2])
      | color('blue')
      | plot(0.35*xp,0.2*yp)
  Line194 : PMComponent  Tag=PSATblock  Description=Power Flow  PhysicalDomain=psatdomain  LeftPortType=p1  RightPortType=p1  LConnTagsString=__newl0  RConnTagsString=__newr0  mask(Line){p3_4_5q=[100  115  60], p6q=82.89, p8q=[0.125], p9q=[0.000994719], p10q=[0.007460394e-6], p13_14_15q=[0.0 0.0 0.0], p16q=on}
      mask prompts: p3_4_5q "Power, Voltage and Frequency Ratings [MVA, kV, Hz]"; p6q "Length of line [km] (0 for p.u. parameters)"; p8q "Resistance [p.u. (Ohms/km)]"; p9q "Reactance [p.u. (H/km)]"; p10q "Susceptance [p.u. (F/km)]"; p13_14_15q "Imax, Pmax and Smax [p.u., p.u., p.u.]"; p16q "Connected"
      mask help: This block defines a pi model for a tree phase line.
      mask init:
      | [xp,yp] = fm_draw('pi');
      mask CallbackString: ||||||fm_block
      mask Display:
      | plot([-1  1  1 -1 -1],[-0.2 -0.2 0.2 0.2 -0.2])
      | color('blue')
      | plot(0.35*xp,0.2*yp)
  Line195 : PMComponent  Tag=PSATblock  Description=Power Flow  PhysicalDomain=psatdomain  LeftPortType=p1  RightPortType=p1  LConnTagsString=__newl0  RConnTagsString=__newr0  mask(Line){p3_4_5q=[100  115  60], p6q=6.6, p8q=[0.125], p9q=[0.000994719], p10q=[0.007460394e-6], p13_14_15q=[0.0 0.0 0.0], p16q=on}
      mask prompts: p3_4_5q "Power, Voltage and Frequency Ratings [MVA, kV, Hz]"; p6q "Length of line [km] (0 for p.u. parameters)"; p8q "Resistance [p.u. (Ohms/km)]"; p9q "Reactance [p.u. (H/km)]"; p10q "Susceptance [p.u. (F/km)]"; p13_14_15q "Imax, Pmax and Smax [p.u., p.u., p.u.]"; p16q "Connected"
      mask help: This block defines a pi model for a tree phase line.
      mask init:
      | [xp,yp] = fm_draw('pi');
      mask CallbackString: ||||||fm_block
      mask Display:
      | plot([-1  1  1 -1 -1],[-0.2 -0.2 0.2 0.2 -0.2])
      | color('blue')
      | plot(0.35*xp,0.2*yp)
  Line196 : PMComponent  Tag=PSATblock  Description=Power Flow  PhysicalDomain=psatdomain  LeftPortType=p1  RightPortType=p1  LConnTagsString=__newl0  RConnTagsString=__newr0  mask(Line){p3_4_5q=[100  115  60], p6q=26.56, p8q=[0.125], p9q=[0.000994719], p10q=[0.007460394e-6], p13_14_15q=[0.0 0.0 0.0], p16q=on}
      mask prompts: p3_4_5q "Power, Voltage and Frequency Ratings [MVA, kV, Hz]"; p6q "Length of line [km] (0 for p.u. parameters)"; p8q "Resistance [p.u. (Ohms/km)]"; p9q "Reactance [p.u. (H/km)]"; p10q "Susceptance [p.u. (F/km)]"; p13_14_15q "Imax, Pmax and Smax [p.u., p.u., p.u.]"; p16q "Connected"
      mask help: This block defines a pi model for a tree phase line.
      mask init:
      | [xp,yp] = fm_draw('pi');
      mask CallbackString: ||||||fm_block
      mask Display:
      | plot([-1  1  1 -1 -1],[-0.2 -0.2 0.2 0.2 -0.2])
      | color('blue')
      | plot(0.35*xp,0.2*yp)
  Line197 : PMComponent  Tag=PSATblock  Description=Power Flow  PhysicalDomain=psatdomain  LeftPortType=p1  RightPortType=p1  LConnTagsString=__newl0  RConnTagsString=__newr0  mask(Line){p3_4_5q=[100  115  60], p6q=51.36, p8q=[0.125], p9q=[0.000994719], p10q=[0.007460394e-6], p13_14_15q=[0.0 0.0 0.0], p16q=on}
      mask prompts: p3_4_5q "Power, Voltage and Frequency Ratings [MVA, kV, Hz]"; p6q "Length of line [km] (0 for p.u. parameters)"; p8q "Resistance [p.u. (Ohms/km)]"; p9q "Reactance [p.u. (H/km)]"; p10q "Susceptance [p.u. (F/km)]"; p13_14_15q "Imax, Pmax and Smax [p.u., p.u., p.u.]"; p16q "Connected"
      mask help: This block defines a pi model for a tree phase line.
      mask init:
      | [xp,yp] = fm_draw('pi');
      mask CallbackString: ||||||fm_block
      mask Display:
      | plot([-1  1  1 -1 -1],[-0.2 -0.2 0.2 0.2 -0.2])
      | color('blue')
      | plot(0.35*xp,0.2*yp)
  Line198 : PMComponent  Tag=PSATblock  Description=Power Flow  PhysicalDomain=psatdomain  LeftPortType=p1  RightPortType=p1  LConnTagsString=__newl0  RConnTagsString=__newr0  mask(Line){p3_4_5q=[100  115  60], p6q=17.67, p8q=[0.125], p9q=[0.000994719], p10q=[0.007460394e-6], p13_14_15q=[0.0 0.0 0.0], p16q=on}
      mask prompts: p3_4_5q "Power, Voltage and Frequency Ratings [MVA, kV, Hz]"; p6q "Length of line [km] (0 for p.u. parameters)"; p8q "Resistance [p.u. (Ohms/km)]"; p9q "Reactance [p.u. (H/km)]"; p10q "Susceptance [p.u. (F/km)]"; p13_14_15q "Imax, Pmax and Smax [p.u., p.u., p.u.]"; p16q "Connected"
      mask help: This block defines a pi model for a tree phase line.
      mask init:
      | [xp,yp] = fm_draw('pi');
      mask CallbackString: ||||||fm_block
      mask Display:
      | plot([-1  1  1 -1 -1],[-0.2 -0.2 0.2 0.2 -0.2])
      | color('blue')
      | plot(0.35*xp,0.2*yp)
  Line199 : PMComponent  Tag=PSATblock  Description=Power Flow  PhysicalDomain=psatdomain  LeftPortType=p1  RightPortType=p1  LConnTagsString=__newl0  RConnTagsString=__newr0  mask(Line){p3_4_5q=[100  115  60], p6q=24.80, p8q=[0.125], p9q=[0.000994719], p10q=[0.007460394e-6], p13_14_15q=[0.0 0.0 0.0], p16q=on}
      mask prompts: p3_4_5q "Power, Voltage and Frequency Ratings [MVA, kV, Hz]"; p6q "Length of line [km] (0 for p.u. parameters)"; p8q "Resistance [p.u. (Ohms/km)]"; p9q "Reactance [p.u. (H/km)]"; p10q "Susceptance [p.u. (F/km)]"; p13_14_15q "Imax, Pmax and Smax [p.u., p.u., p.u.]"; p16q "Connected"
      mask help: This block defines a pi model for a tree phase line.
      mask init:
      | [xp,yp] = fm_draw('pi');
      mask CallbackString: ||||||fm_block
      mask Display:
      | plot([-1  1  1 -1 -1],[-0.2 -0.2 0.2 0.2 -0.2])
      | color('blue')
      | plot(0.35*xp,0.2*yp)
  Line2 : PMComponent  Tag=PSATblock  Description=Power Flow  PhysicalDomain=psatdomain  LeftPortType=p1  RightPortType=p1  LConnTagsString=__newl0  RConnTagsString=__newr0  mask(Line){p3_4_5q=[100 765 60], p6q=[161], p8q=[0.012], p9q=[0.0008727], p10q=[0.013204566e-6], p13_14_15q=[25.29 22.76 25.29], p16q=on}
      mask prompts: p3_4_5q "Power, Voltage and Frequency Ratings [MVA, kV, Hz]"; p6q "Length of line [km] (0 for p.u. parameters)"; p8q "Resistance [p.u. (Ohms/km)]"; p9q "Reactance [p.u. (H/km)]"; p10q "Susceptance [p.u. (F/km)]"; p13_14_15q "Imax, Pmax and Smax [p.u., p.u., p.u.]"; p16q "Connected"
      mask help: This block defines a pi model for a tree phase line.
      mask init:
      | [xp,yp] = fm_draw('pi');
      mask CallbackString: ||||||fm_block
      mask Display:
      | plot([-1  1  1 -1 -1],[-0.2 -0.2 0.2 0.2 -0.2])
      | color('blue')
      | plot(0.35*xp,0.2*yp)
  Line20 : PMComponent  Tag=PSATblock  Description=Power Flow  PhysicalDomain=psatdomain  LeftPortType=p1  RightPortType=p1  LConnTagsString=__newl0  RConnTagsString=__newr0  mask(Line){p3_4_5q=[100  400  60], p6q=164, p8q=[0.033806452], p9q=[0.000933966], p10q=[0.012626303e-6], p13_14_15q=[30.5 27.7 30.5], p16q=on}
      mask prompts: p3_4_5q "Power, Voltage and Frequency Ratings [MVA, kV, Hz]"; p6q "Length of line [km] (0 for p.u. parameters)"; p8q "Resistance [p.u. (Ohms/km)]"; p9q "Reactance [p.u. (H/km)]"; p10q "Susceptance [p.u. (F/km)]"; p13_14_15q "Imax, Pmax and Smax [p.u., p.u., p.u.]"; p16q "Connected"
      mask help: This block defines a pi model for a tree phase line.
      mask init:
      | [xp,yp] = fm_draw('pi');
      mask CallbackString: ||||||fm_block
      mask Display:
      | plot([-1  1  1 -1 -1],[-0.2 -0.2 0.2 0.2 -0.2])
      | color('blue')
      | plot(0.35*xp,0.2*yp)
  Line200 : PMComponent  Tag=PSATblock  Description=Power Flow  PhysicalDomain=psatdomain  LeftPortType=p1  RightPortType=p1  LConnTagsString=__newl0  RConnTagsString=__newr0  mask(Line){p3_4_5q=[100  115  60], p6q=7.55, p8q=[0.125], p9q=[0.000994719], p10q=[0.007460394e-6], p13_14_15q=[0.0 0.0 0.0], p16q=on}
      mask prompts: p3_4_5q "Power, Voltage and Frequency Ratings [MVA, kV, Hz]"; p6q "Length of line [km] (0 for p.u. parameters)"; p8q "Resistance [p.u. (Ohms/km)]"; p9q "Reactance [p.u. (H/km)]"; p10q "Susceptance [p.u. (F/km)]"; p13_14_15q "Imax, Pmax and Smax [p.u., p.u., p.u.]"; p16q "Connected"
      mask help: This block defines a pi model for a tree phase line.
      mask init:
      | [xp,yp] = fm_draw('pi');
      mask CallbackString: ||||||fm_block
      mask Display:
      | plot([-1  1  1 -1 -1],[-0.2 -0.2 0.2 0.2 -0.2])
      | color('blue')
      | plot(0.35*xp,0.2*yp)
  Line201 : PMComponent  Tag=PSATblock  Description=Power Flow  PhysicalDomain=psatdomain  LeftPortType=p1  RightPortType=p1  LConnTagsString=__newl0  RConnTagsString=__newr0  mask(Line){p3_4_5q=[100  115  60], p6q=7.15, p8q=[0.125], p9q=[0.000994719], p10q=[0.007460394e-6], p13_14_15q=[0.0 0.0 0.0], p16q=on}
      mask prompts: p3_4_5q "Power, Voltage and Frequency Ratings [MVA, kV, Hz]"; p6q "Length of line [km] (0 for p.u. parameters)"; p8q "Resistance [p.u. (Ohms/km)]"; p9q "Reactance [p.u. (H/km)]"; p10q "Susceptance [p.u. (F/km)]"; p13_14_15q "Imax, Pmax and Smax [p.u., p.u., p.u.]"; p16q "Connected"
      mask help: This block defines a pi model for a tree phase line.
      mask init:
      | [xp,yp] = fm_draw('pi');
      mask CallbackString: ||||||fm_block
      mask Display:
      | plot([-1  1  1 -1 -1],[-0.2 -0.2 0.2 0.2 -0.2])
      | color('blue')
      | plot(0.35*xp,0.2*yp)
  Line202 : PMComponent  Tag=PSATblock  Description=Power Flow  PhysicalDomain=psatdomain  LeftPortType=p1  RightPortType=p1  LConnTagsString=__newl0  RConnTagsString=__newr0  mask(Line){p3_4_5q=[100  115  60], p6q=7.93, p8q=[0.125], p9q=[0.000994719], p10q=[0.007460394e-6], p13_14_15q=[0.0 0.0 0.0], p16q=on}
      mask prompts: p3_4_5q "Power, Voltage and Frequency Ratings [MVA, kV, Hz]"; p6q "Length of line [km] (0 for p.u. parameters)"; p8q "Resistance [p.u. (Ohms/km)]"; p9q "Reactance [p.u. (H/km)]"; p10q "Susceptance [p.u. (F/km)]"; p13_14_15q "Imax, Pmax and Smax [p.u., p.u., p.u.]"; p16q "Connected"
      mask help: This block defines a pi model for a tree phase line.
      mask init:
      | [xp,yp] = fm_draw('pi');
      mask CallbackString: ||||||fm_block
      mask Display:
      | plot([-1  1  1 -1 -1],[-0.2 -0.2 0.2 0.2 -0.2])
      | color('blue')
      | plot(0.35*xp,0.2*yp)
  Line203 : PMComponent  Tag=PSATblock  Description=Power Flow  PhysicalDomain=psatdomain  LeftPortType=p1  RightPortType=p1  LConnTagsString=__newl0  RConnTagsString=__newr0  mask(Line){p3_4_5q=[100  115  60], p6q=12.43, p8q=[0.125], p9q=[0.000994719], p10q=[0.007460394e-6], p13_14_15q=[0.0 0.0 0.0], p16q=on}
      mask prompts: p3_4_5q "Power, Voltage and Frequency Ratings [MVA, kV, Hz]"; p6q "Length of line [km] (0 for p.u. parameters)"; p8q "Resistance [p.u. (Ohms/km)]"; p9q "Reactance [p.u. (H/km)]"; p10q "Susceptance [p.u. (F/km)]"; p13_14_15q "Imax, Pmax and Smax [p.u., p.u., p.u.]"; p16q "Connected"
      mask help: This block defines a pi model for a tree phase line.
      mask init:
      | [xp,yp] = fm_draw('pi');
      mask CallbackString: ||||||fm_block
      mask Display:
      | plot([-1  1  1 -1 -1],[-0.2 -0.2 0.2 0.2 -0.2])
      | color('blue')
      | plot(0.35*xp,0.2*yp)
  Line204 : PMComponent  Tag=PSATblock  Description=Power Flow  PhysicalDomain=psatdomain  LeftPortType=p1  RightPortType=p1  LConnTagsString=__newl0  RConnTagsString=__newr0  mask(Line){p3_4_5q=[100  115  60], p6q=29.66, p8q=[0.125], p9q=[0.000994719], p10q=[0.007460394e-6], p13_14_15q=[0.0 0.0 0.0], p16q=on}
      mask prompts: p3_4_5q "Power, Voltage and Frequency Ratings [MVA, kV, Hz]"; p6q "Length of line [km] (0 for p.u. parameters)"; p8q "Resistance [p.u. (Ohms/km)]"; p9q "Reactance [p.u. (H/km)]"; p10q "Susceptance [p.u. (F/km)]"; p13_14_15q "Imax, Pmax and Smax [p.u., p.u., p.u.]"; p16q "Connected"
      mask help: This block defines a pi model for a tree phase line.
      mask init:
      | [xp,yp] = fm_draw('pi');
      mask CallbackString: ||||||fm_block
      mask Display:
      | plot([-1  1  1 -1 -1],[-0.2 -0.2 0.2 0.2 -0.2])
      | color('blue')
      | plot(0.35*xp,0.2*yp)
  Line205 : PMComponent  Tag=PSATblock  Description=Power Flow  PhysicalDomain=psatdomain  LeftPortType=p1  RightPortType=p1  LConnTagsString=__newl0  RConnTagsString=__newr0  mask(Line){p3_4_5q=[100  115  60], p6q=57.04, p8q=[0.125], p9q=[0.000994719], p10q=[0.007460394e-6], p13_14_15q=[0.0 0.0 0.0], p16q=on}
      mask prompts: p3_4_5q "Power, Voltage and Frequency Ratings [MVA, kV, Hz]"; p6q "Length of line [km] (0 for p.u. parameters)"; p8q "Resistance [p.u. (Ohms/km)]"; p9q "Reactance [p.u. (H/km)]"; p10q "Susceptance [p.u. (F/km)]"; p13_14_15q "Imax, Pmax and Smax [p.u., p.u., p.u.]"; p16q "Connected"
      mask help: This block defines a pi model for a tree phase line.
      mask init:
      | [xp,yp] = fm_draw('pi');
      mask CallbackString: ||||||fm_block
      mask Display:
      | plot([-1  1  1 -1 -1],[-0.2 -0.2 0.2 0.2 -0.2])
      | color('blue')
      | plot(0.35*xp,0.2*yp)
  Line206 : PMComponent  Tag=PSATblock  Description=Power Flow  PhysicalDomain=psatdomain  LeftPortType=p1  RightPortType=p1  LConnTagsString=__newl0  RConnTagsString=__newr0  mask(Line){p3_4_5q=[100  115  60], p6q=35.54, p8q=[0.125], p9q=[0.000994719], p10q=[0.007460394e-6], p13_14_15q=[0.0 0.0 0.0], p16q=on}
      mask prompts: p3_4_5q "Power, Voltage and Frequency Ratings [MVA, kV, Hz]"; p6q "Length of line [km] (0 for p.u. parameters)"; p8q "Resistance [p.u. (Ohms/km)]"; p9q "Reactance [p.u. (H/km)]"; p10q "Susceptance [p.u. (F/km)]"; p13_14_15q "Imax, Pmax and Smax [p.u., p.u., p.u.]"; p16q "Connected"
      mask help: This block defines a pi model for a tree phase line.
      mask init:
      | [xp,yp] = fm_draw('pi');
      mask CallbackString: ||||||fm_block
      mask Display:
      | plot([-1  1  1 -1 -1],[-0.2 -0.2 0.2 0.2 -0.2])
      | color('blue')
      | plot(0.35*xp,0.2*yp)
  Line207 : PMComponent  Tag=PSATblock  Description=Power Flow  PhysicalDomain=psatdomain  LeftPortType=p1  RightPortType=p1  LConnTagsString=__newl0  RConnTagsString=__newr0  mask(Line){p3_4_5q=[100  115  60], p6q=62.09, p8q=[0.125], p9q=[0.000994719], p10q=[0.007460394e-6], p13_14_15q=[0.0 0.0 0.0], p16q=on}
      mask prompts: p3_4_5q "Power, Voltage and Frequency Ratings [MVA, kV, Hz]"; p6q "Length of line [km] (0 for p.u. parameters)"; p8q "Resistance [p.u. (Ohms/km)]"; p9q "Reactance [p.u. (H/km)]"; p10q "Susceptance [p.u. (F/km)]"; p13_14_15q "Imax, Pmax and Smax [p.u., p.u., p.u.]"; p16q "Connected"
      mask help: This block defines a pi model for a tree phase line.
      mask init:
      | [xp,yp] = fm_draw('pi');
      mask CallbackString: ||||||fm_block
      mask Display:
      | plot([-1  1  1 -1 -1],[-0.2 -0.2 0.2 0.2 -0.2])
      | color('blue')
      | plot(0.35*xp,0.2*yp)
  Line208 : PMComponent  Tag=PSATblock  Description=Power Flow  PhysicalDomain=psatdomain  LeftPortType=p1  RightPortType=p1  LConnTagsString=__newl0  RConnTagsString=__newr0  mask(Line){p3_4_5q=[100  115  60], p6q=147.84, p8q=[0.125], p9q=[0.000994719], p10q=[0.007460394e-6], p13_14_15q=[0.0 0.0 0.0], p16q=on}
      mask prompts: p3_4_5q "Power, Voltage and Frequency Ratings [MVA, kV, Hz]"; p6q "Length of line [km] (0 for p.u. parameters)"; p8q "Resistance [p.u. (Ohms/km)]"; p9q "Reactance [p.u. (H/km)]"; p10q "Susceptance [p.u. (F/km)]"; p13_14_15q "Imax, Pmax and Smax [p.u., p.u., p.u.]"; p16q "Connected"
      mask help: This block defines a pi model for a tree phase line.
      mask init:
      | [xp,yp] = fm_draw('pi');
      mask CallbackString: ||||||fm_block
      mask Display:
      | plot([-1  1  1 -1 -1],[-0.2 -0.2 0.2 0.2 -0.2])
      | color('blue')
      | plot(0.35*xp,0.2*yp)
  Line209 : PMComponent  Tag=PSATblock  Description=Power Flow  PhysicalDomain=psatdomain  LeftPortType=p1  RightPortType=p1  LConnTagsString=__newl0  RConnTagsString=__newr0  mask(Line){p3_4_5q=[100  115  60], p6q=96.28, p8q=[0.125], p9q=[0.000994719], p10q=[0.007460394e-6], p13_14_15q=[0.0 0.0 0.0], p16q=on}
      mask prompts: p3_4_5q "Power, Voltage and Frequency Ratings [MVA, kV, Hz]"; p6q "Length of line [km] (0 for p.u. parameters)"; p8q "Resistance [p.u. (Ohms/km)]"; p9q "Reactance [p.u. (H/km)]"; p10q "Susceptance [p.u. (F/km)]"; p13_14_15q "Imax, Pmax and Smax [p.u., p.u., p.u.]"; p16q "Connected"
      mask help: This block defines a pi model for a tree phase line.
      mask init:
      | [xp,yp] = fm_draw('pi');
      mask CallbackString: ||||||fm_block
      mask Display:
      | plot([-1  1  1 -1 -1],[-0.2 -0.2 0.2 0.2 -0.2])
      | color('blue')
      | plot(0.35*xp,0.2*yp)
  Line21 : PMComponent  Tag=PSATblock  Description=Power Flow  PhysicalDomain=psatdomain  LeftPortType=p1  RightPortType=p1  LConnTagsString=__newl0  RConnTagsString=__newr0  mask(Line){p3_4_5q=[100  230  60], p6q=7, p8q=[0.05], p9q=[0.001294461], p10q=[0.008941863e-6], p13_14_15q=[170 155 170], p16q=on}
      mask prompts: p3_4_5q "Power, Voltage and Frequency Ratings [MVA, kV, Hz]"; p6q "Length of line [km] (0 for p.u. parameters)"; p8q "Resistance [p.u. (Ohms/km)]"; p9q "Reactance [p.u. (H/km)]"; p10q "Susceptance [p.u. (F/km)]"; p13_14_15q "Imax, Pmax and Smax [p.u., p.u., p.u.]"; p16q "Connected"
      mask help: This block defines a pi model for a tree phase line.
      mask init:
      | [xp,yp] = fm_draw('pi');
      mask CallbackString: ||||||fm_block
      mask Display:
      | plot([-1  1  1 -1 -1],[-0.2 -0.2 0.2 0.2 -0.2])
      | color('blue')
      | plot(0.35*xp,0.2*yp)
  Line210 : PMComponent  Tag=PSATblock  Description=Power Flow  PhysicalDomain=psatdomain  LeftPortType=p1  RightPortType=p1  LConnTagsString=__newl0  RConnTagsString=__newr0  mask(Line){p3_4_5q=[100  115  60], p6q=78.19, p8q=[0.125], p9q=[0.000994719], p10q=[0.007460394e-6], p13_14_15q=[0.0 0.0 0.0], p16q=on}
      mask prompts: p3_4_5q "Power, Voltage and Frequency Ratings [MVA, kV, Hz]"; p6q "Length of line [km] (0 for p.u. parameters)"; p8q "Resistance [p.u. (Ohms/km)]"; p9q "Reactance [p.u. (H/km)]"; p10q "Susceptance [p.u. (F/km)]"; p13_14_15q "Imax, Pmax and Smax [p.u., p.u., p.u.]"; p16q "Connected"
      mask help: This block defines a pi model for a tree phase line.
      mask init:
      | [xp,yp] = fm_draw('pi');
      mask CallbackString: ||||||fm_block
      mask Display:
      | plot([-1  1  1 -1 -1],[-0.2 -0.2 0.2 0.2 -0.2])
      | color('blue')
      | plot(0.35*xp,0.2*yp)
  Line211 : PMComponent  Tag=PSATblock  Description=Power Flow  PhysicalDomain=psatdomain  LeftPortType=p1  RightPortType=p1  LConnTagsString=__newl0  RConnTagsString=__newr0  mask(Line){p3_4_5q=[100  115  60], p6q=42.63, p8q=[0.125], p9q=[0.000994719], p10q=[0.007460394e-6], p13_14_15q=[0.0 0.0 0.0], p16q=on}
      mask prompts: p3_4_5q "Power, Voltage and Frequency Ratings [MVA, kV, Hz]"; p6q "Length of line [km] (0 for p.u. parameters)"; p8q "Resistance [p.u. (Ohms/km)]"; p9q "Reactance [p.u. (H/km)]"; p10q "Susceptance [p.u. (F/km)]"; p13_14_15q "Imax, Pmax and Smax [p.u., p.u., p.u.]"; p16q "Connected"
      mask help: This block defines a pi model for a tree phase line.
      mask init:
      | [xp,yp] = fm_draw('pi');
      mask CallbackString: ||||||fm_block
      mask Display:
      | plot([-1  1  1 -1 -1],[-0.2 -0.2 0.2 0.2 -0.2])
      | color('blue')
      | plot(0.35*xp,0.2*yp)
  Line212 : PMComponent  Tag=PSATblock  Description=Power Flow  PhysicalDomain=psatdomain  LeftPortType=p1  RightPortType=p1  LConnTagsString=__newl0  RConnTagsString=__newr0  mask(Line){p3_4_5q=[100  115  60], p6q=30.96, p8q=[0.125], p9q=[0.000994719], p10q=[0.007460394e-6], p13_14_15q=[0.0 0.0 0.0], p16q=on}
      mask prompts: p3_4_5q "Power, Voltage and Frequency Ratings [MVA, kV, Hz]"; p6q "Length of line [km] (0 for p.u. parameters)"; p8q "Resistance [p.u. (Ohms/km)]"; p9q "Reactance [p.u. (H/km)]"; p10q "Susceptance [p.u. (F/km)]"; p13_14_15q "Imax, Pmax and Smax [p.u., p.u., p.u.]"; p16q "Connected"
      mask help: This block defines a pi model for a tree phase line.
      mask init:
      | [xp,yp] = fm_draw('pi');
      mask CallbackString: ||||||fm_block
      mask Display:
      | plot([-1  1  1 -1 -1],[-0.2 -0.2 0.2 0.2 -0.2])
      | color('blue')
      | plot(0.35*xp,0.2*yp)
  Line213 : PMComponent  Tag=PSATblock  Description=Power Flow  PhysicalDomain=psatdomain  LeftPortType=p1  RightPortType=p1  LConnTagsString=__newl0  RConnTagsString=__newr0  mask(Line){p3_4_5q=[100  115  60], p6q=71.84, p8q=[0.125], p9q=[0.000994719], p10q=[0.007460394e-6], p13_14_15q=[0.0 0.0 0.0], p16q=on}
      mask prompts: p3_4_5q "Power, Voltage and Frequency Ratings [MVA, kV, Hz]"; p6q "Length of line [km] (0 for p.u. parameters)"; p8q "Resistance [p.u. (Ohms/km)]"; p9q "Reactance [p.u. (H/km)]"; p10q "Susceptance [p.u. (F/km)]"; p13_14_15q "Imax, Pmax and Smax [p.u., p.u., p.u.]"; p16q "Connected"
      mask help: This block defines a pi model for a tree phase line.
      mask init:
      | [xp,yp] = fm_draw('pi');
      mask CallbackString: ||||||fm_block
      mask Display:
      | plot([-1  1  1 -1 -1],[-0.2 -0.2 0.2 0.2 -0.2])
      | color('blue')
      | plot(0.35*xp,0.2*yp)
  Line214 : PMComponent  Tag=PSATblock  Description=Power Flow  PhysicalDomain=psatdomain  LeftPortType=p1  RightPortType=p1  LConnTagsString=__newl0  RConnTagsString=__newr0  mask(Line){p3_4_5q=[100  115  60], p6q=48.68, p8q=[0.125], p9q=[0.000994719], p10q=[0.007460394e-6], p13_14_15q=[0.0 0.0 0.0], p16q=on}
      mask prompts: p3_4_5q "Power, Voltage and Frequency Ratings [MVA, kV, Hz]"; p6q "Length of line [km] (0 for p.u. parameters)"; p8q "Resistance [p.u. (Ohms/km)]"; p9q "Reactance [p.u. (H/km)]"; p10q "Susceptance [p.u. (F/km)]"; p13_14_15q "Imax, Pmax and Smax [p.u., p.u., p.u.]"; p16q "Connected"
      mask help: This block defines a pi model for a tree phase line.
      mask init:
      | [xp,yp] = fm_draw('pi');
      mask CallbackString: ||||||fm_block
      mask Display:
      | plot([-1  1  1 -1 -1],[-0.2 -0.2 0.2 0.2 -0.2])
      | color('blue')
      | plot(0.35*xp,0.2*yp)
  Line215 : PMComponent  Tag=PSATblock  Description=Power Flow  PhysicalDomain=psatdomain  LeftPortType=p1  RightPortType=p1  LConnTagsString=__newl0  RConnTagsString=__newr0  mask(Line){p3_4_5q=[100  115  60], p6q=30.16, p8q=[0.125], p9q=[0.000994719], p10q=[0.007460394e-6], p13_14_15q=[0.0 0.0 0.0], p16q=on}
      mask prompts: p3_4_5q "Power, Voltage and Frequency Ratings [MVA, kV, Hz]"; p6q "Length of line [km] (0 for p.u. parameters)"; p8q "Resistance [p.u. (Ohms/km)]"; p9q "Reactance [p.u. (H/km)]"; p10q "Susceptance [p.u. (F/km)]"; p13_14_15q "Imax, Pmax and Smax [p.u., p.u., p.u.]"; p16q "Connected"
      mask help: This block defines a pi model for a tree phase line.
      mask init:
      | [xp,yp] = fm_draw('pi');
      mask CallbackString: ||||||fm_block
      mask Display:
      | plot([-1  1  1 -1 -1],[-0.2 -0.2 0.2 0.2 -0.2])
      | color('blue')
      | plot(0.35*xp,0.2*yp)
  Line216 : PMComponent  Tag=PSATblock  Description=Power Flow  PhysicalDomain=psatdomain  LeftPortType=p1  RightPortType=p1  LConnTagsString=__newl0  RConnTagsString=__newr0  mask(Line){p3_4_5q=[100  115  60], p6q=22.69, p8q=[0.125], p9q=[0.000994719], p10q=[0.007460394e-6], p13_14_15q=[0.0 0.0 0.0], p16q=on}
      mask prompts: p3_4_5q "Power, Voltage and Frequency Ratings [MVA, kV, Hz]"; p6q "Length of line [km] (0 for p.u. parameters)"; p8q "Resistance [p.u. (Ohms/km)]"; p9q "Reactance [p.u. (H/km)]"; p10q "Susceptance [p.u. (F/km)]"; p13_14_15q "Imax, Pmax and Smax [p.u., p.u., p.u.]"; p16q "Connected"
      mask help: This block defines a pi model for a tree phase line.
      mask init:
      | [xp,yp] = fm_draw('pi');
      mask CallbackString: ||||||fm_block
      mask Display:
      | plot([-1  1  1 -1 -1],[-0.2 -0.2 0.2 0.2 -0.2])
      | color('blue')
      | plot(0.35*xp,0.2*yp)
  Line217 : PMComponent  Tag=PSATblock  Description=Power Flow  PhysicalDomain=psatdomain  LeftPortType=p1  RightPortType=p1  LConnTagsString=__newl0  RConnTagsString=__newr0  mask(Line){p3_4_5q=[100  115  60], p6q=78.79, p8q=[0.125], p9q=[0.000994719], p10q=[0.007460394e-6], p13_14_15q=[0.0 0.0 0.0], p16q=on}
      mask prompts: p3_4_5q "Power, Voltage and Frequency Ratings [MVA, kV, Hz]"; p6q "Length of line [km] (0 for p.u. parameters)"; p8q "Resistance [p.u. (Ohms/km)]"; p9q "Reactance [p.u. (H/km)]"; p10q "Susceptance [p.u. (F/km)]"; p13_14_15q "Imax, Pmax and Smax [p.u., p.u., p.u.]"; p16q "Connected"
      mask help: This block defines a pi model for a tree phase line.
      mask init:
      | [xp,yp] = fm_draw('pi');
      mask CallbackString: ||||||fm_block
      mask Display:
      | plot([-1  1  1 -1 -1],[-0.2 -0.2 0.2 0.2 -0.2])
      | color('blue')
      | plot(0.35*xp,0.2*yp)
  Line218 : PMComponent  Tag=PSATblock  Description=Power Flow  PhysicalDomain=psatdomain  LeftPortType=p1  RightPortType=p1  LConnTagsString=__newl0  RConnTagsString=__newr0  mask(Line){p3_4_5q=[100  115  60], p6q=48.91, p8q=[0.125], p9q=[0.000994719], p10q=[0.007460394e-6], p13_14_15q=[0.0 0.0 0.0], p16q=on}
      mask prompts: p3_4_5q "Power, Voltage and Frequency Ratings [MVA, kV, Hz]"; p6q "Length of line [km] (0 for p.u. parameters)"; p8q "Resistance [p.u. (Ohms/km)]"; p9q "Reactance [p.u. (H/km)]"; p10q "Susceptance [p.u. (F/km)]"; p13_14_15q "Imax, Pmax and Smax [p.u., p.u., p.u.]"; p16q "Connected"
      mask help: This block defines a pi model for a tree phase line.
      mask init:
      | [xp,yp] = fm_draw('pi');
      mask CallbackString: ||||||fm_block
      mask Display:
      | plot([-1  1  1 -1 -1],[-0.2 -0.2 0.2 0.2 -0.2])
      | color('blue')
      | plot(0.35*xp,0.2*yp)
  Line219 : PMComponent  Tag=PSATblock  Description=Power Flow  PhysicalDomain=psatdomain  LeftPortType=p1  RightPortType=p1  LConnTagsString=__newl0  RConnTagsString=__newr0  mask(Line){p3_4_5q=[100  115  60], p6q=25.79, p8q=[0.125], p9q=[0.000994719], p10q=[0.007460394e-6], p13_14_15q=[0.0 0.0 0.0], p16q=on}
      mask prompts: p3_4_5q "Power, Voltage and Frequency Ratings [MVA, kV, Hz]"; p6q "Length of line [km] (0 for p.u. parameters)"; p8q "Resistance [p.u. (Ohms/km)]"; p9q "Reactance [p.u. (H/km)]"; p10q "Susceptance [p.u. (F/km)]"; p13_14_15q "Imax, Pmax and Smax [p.u., p.u., p.u.]"; p16q "Connected"
      mask help: This block defines a pi model for a tree phase line.
      mask init:
      | [xp,yp] = fm_draw('pi');
      mask CallbackString: ||||||fm_block
      mask Display:
      | plot([-1  1  1 -1 -1],[-0.2 -0.2 0.2 0.2 -0.2])
      | color('blue')
      | plot(0.35*xp,0.2*yp)
  Line22 : PMComponent  Tag=PSATblock  Description=Power Flow  PhysicalDomain=psatdomain  LeftPortType=p1  RightPortType=p1  LConnTagsString=__newl0  RConnTagsString=__newr0  mask(Line){p3_4_5q=[100  400  60], p6q=210, p8q=[0.033806452], p9q=[0.000933966], p10q=[0.012626303e-6], p13_14_15q=[23.8 21.6 23.8], p16q=on}
      mask prompts: p3_4_5q "Power, Voltage and Frequency Ratings [MVA, kV, Hz]"; p6q "Length of line [km] (0 for p.u. parameters)"; p8q "Resistance [p.u. (Ohms/km)]"; p9q "Reactance [p.u. (H/km)]"; p10q "Susceptance [p.u. (F/km)]"; p13_14_15q "Imax, Pmax and Smax [p.u., p.u., p.u.]"; p16q "Connected"
      mask help: This block defines a pi model for a tree phase line.
      mask init:
      | [xp,yp] = fm_draw('pi');
      mask CallbackString: ||||||fm_block
      mask Display:
      | plot([-1  1  1 -1 -1],[-0.2 -0.2 0.2 0.2 -0.2])
      | color('blue')
      | plot(0.35*xp,0.2*yp)
  Line220 : PMComponent  Tag=PSATblock  Description=Power Flow  PhysicalDomain=psatdomain  LeftPortType=p1  RightPortType=p1  LConnTagsString=__newl0  RConnTagsString=__newr0  mask(Line){p3_4_5q=[100  115  60], p6q=25.79, p8q=[0.125], p9q=[0.000994719], p10q=[0.007460394e-6], p13_14_15q=[0.0 0.0 0.0], p16q=on}
      mask prompts: p3_4_5q "Power, Voltage and Frequency Ratings [MVA, kV, Hz]"; p6q "Length of line [km] (0 for p.u. parameters)"; p8q "Resistance [p.u. (Ohms/km)]"; p9q "Reactance [p.u. (H/km)]"; p10q "Susceptance [p.u. (F/km)]"; p13_14_15q "Imax, Pmax and Smax [p.u., p.u., p.u.]"; p16q "Connected"
      mask help: This block defines a pi model for a tree phase line.
      mask init:
      | [xp,yp] = fm_draw('pi');
      mask CallbackString: ||||||fm_block
      mask Display:
      | plot([-1  1  1 -1 -1],[-0.2 -0.2 0.2 0.2 -0.2])
      | color('blue')
      | plot(0.35*xp,0.2*yp)
  Line221 : PMComponent  Tag=PSATblock  Description=Power Flow  PhysicalDomain=psatdomain  LeftPortType=p1  RightPortType=p1  LConnTagsString=__newl0  RConnTagsString=__newr0  mask(Line){p3_4_5q=[100  115  60], p6q=21.21, p8q=[0.125], p9q=[0.000994719], p10q=[0.007460394e-6], p13_14_15q=[0.0 0.0 0.0], p16q=on}
      mask prompts: p3_4_5q "Power, Voltage and Frequency Ratings [MVA, kV, Hz]"; p6q "Length of line [km] (0 for p.u. parameters)"; p8q "Resistance [p.u. (Ohms/km)]"; p9q "Reactance [p.u. (H/km)]"; p10q "Susceptance [p.u. (F/km)]"; p13_14_15q "Imax, Pmax and Smax [p.u., p.u., p.u.]"; p16q "Connected"
      mask help: This block defines a pi model for a tree phase line.
      mask init:
      | [xp,yp] = fm_draw('pi');
      mask CallbackString: ||||||fm_block
      mask Display:
      | plot([-1  1  1 -1 -1],[-0.2 -0.2 0.2 0.2 -0.2])
      | color('blue')
      | plot(0.35*xp,0.2*yp)
  Line222 : PMComponent  Tag=PSATblock  Description=Power Flow  PhysicalDomain=psatdomain  LeftPortType=p1  RightPortType=p1  LConnTagsString=__newl0  RConnTagsString=__newr0  mask(Line){p3_4_5q=[100  115  60], p6q=10, p8q=[0.125], p9q=[0.000994719], p10q=[0.007460394e-6], p13_14_15q=[0.0 0.0 0.0], p16q=on}
      mask prompts: p3_4_5q "Power, Voltage and Frequency Ratings [MVA, kV, Hz]"; p6q "Length of line [km] (0 for p.u. parameters)"; p8q "Resistance [p.u. (Ohms/km)]"; p9q "Reactance [p.u. (H/km)]"; p10q "Susceptance [p.u. (F/km)]"; p13_14_15q "Imax, Pmax and Smax [p.u., p.u., p.u.]"; p16q "Connected"
      mask help: This block defines a pi model for a tree phase line.
      mask init:
      | [xp,yp] = fm_draw('pi');
      mask CallbackString: ||||||fm_block
      mask Display:
      | plot([-1  1  1 -1 -1],[-0.2 -0.2 0.2 0.2 -0.2])
      | color('blue')
      | plot(0.35*xp,0.2*yp)
  Line223 : PMComponent  Tag=PSATblock  Description=Power Flow  PhysicalDomain=psatdomain  LeftPortType=p1  RightPortType=p1  LConnTagsString=__newl0  RConnTagsString=__newr0  mask(Line){p3_4_5q=[100  115  60], p6q=36.26, p8q=[0.125], p9q=[0.000994719], p10q=[0.007460394e-6], p13_14_15q=[0.0 0.0 0.0], p16q=on}
      mask prompts: p3_4_5q "Power, Voltage and Frequency Ratings [MVA, kV, Hz]"; p6q "Length of line [km] (0 for p.u. parameters)"; p8q "Resistance [p.u. (Ohms/km)]"; p9q "Reactance [p.u. (H/km)]"; p10q "Susceptance [p.u. (F/km)]"; p13_14_15q "Imax, Pmax and Smax [p.u., p.u., p.u.]"; p16q "Connected"
      mask help: This block defines a pi model for a tree phase line.
      mask init:
      | [xp,yp] = fm_draw('pi');
      mask CallbackString: ||||||fm_block
      mask Display:
      | plot([-1  1  1 -1 -1],[-0.2 -0.2 0.2 0.2 -0.2])
      | color('blue')
      | plot(0.35*xp,0.2*yp)
  Line224 : PMComponent  Tag=PSATblock  Description=Power Flow  PhysicalDomain=psatdomain  LeftPortType=p1  RightPortType=p1  LConnTagsString=__newl0  RConnTagsString=__newr0  mask(Line){p3_4_5q=[100  115  60], p6q=33.56, p8q=[0.125], p9q=[0.000994719], p10q=[0.007460394e-6], p13_14_15q=[0.0 0.0 0.0], p16q=on}
      mask prompts: p3_4_5q "Power, Voltage and Frequency Ratings [MVA, kV, Hz]"; p6q "Length of line [km] (0 for p.u. parameters)"; p8q "Resistance [p.u. (Ohms/km)]"; p9q "Reactance [p.u. (H/km)]"; p10q "Susceptance [p.u. (F/km)]"; p13_14_15q "Imax, Pmax and Smax [p.u., p.u., p.u.]"; p16q "Connected"
      mask help: This block defines a pi model for a tree phase line.
      mask init:
      | [xp,yp] = fm_draw('pi');
      mask CallbackString: ||||||fm_block
      mask Display:
      | plot([-1  1  1 -1 -1],[-0.2 -0.2 0.2 0.2 -0.2])
      | color('blue')
      | plot(0.35*xp,0.2*yp)
  Line225 : PMComponent  Tag=PSATblock  Description=Power Flow  PhysicalDomain=psatdomain  LeftPortType=p1  RightPortType=p1  LConnTagsString=__newl0  RConnTagsString=__newr0  mask(Line){p3_4_5q=[100  115  60], p6q=39.38, p8q=[0.125], p9q=[0.000994719], p10q=[0.007460394e-6], p13_14_15q=[0.0 0.0 0.0], p16q=on}
      mask prompts: p3_4_5q "Power, Voltage and Frequency Ratings [MVA, kV, Hz]"; p6q "Length of line [km] (0 for p.u. parameters)"; p8q "Resistance [p.u. (Ohms/km)]"; p9q "Reactance [p.u. (H/km)]"; p10q "Susceptance [p.u. (F/km)]"; p13_14_15q "Imax, Pmax and Smax [p.u., p.u., p.u.]"; p16q "Connected"
      mask help: This block defines a pi model for a tree phase line.
      mask init:
      | [xp,yp] = fm_draw('pi');
      mask CallbackString: ||||||fm_block
      mask Display:
      | plot([-1  1  1 -1 -1],[-0.2 -0.2 0.2 0.2 -0.2])
      | color('blue')
      | plot(0.35*xp,0.2*yp)
  Line226 : PMComponent  Tag=PSATblock  Description=Power Flow  PhysicalDomain=psatdomain  LeftPortType=p1  RightPortType=p1  LConnTagsString=__newl0  RConnTagsString=__newr0  mask(Line){p3_4_5q=[100  115  60], p6q=70.12, p8q=[0.125], p9q=[0.000994719], p10q=[0.007460394e-6], p13_14_15q=[0.0 0.0 0.0], p16q=on}
      mask prompts: p3_4_5q "Power, Voltage and Frequency Ratings [MVA, kV, Hz]"; p6q "Length of line [km] (0 for p.u. parameters)"; p8q "Resistance [p.u. (Ohms/km)]"; p9q "Reactance [p.u. (H/km)]"; p10q "Susceptance [p.u. (F/km)]"; p13_14_15q "Imax, Pmax and Smax [p.u., p.u., p.u.]"; p16q "Connected"
      mask help: This block defines a pi model for a tree phase line.
      mask init:
      | [xp,yp] = fm_draw('pi');
      mask CallbackString: ||||||fm_block
      mask Display:
      | plot([-1  1  1 -1 -1],[-0.2 -0.2 0.2 0.2 -0.2])
      | color('blue')
      | plot(0.35*xp,0.2*yp)
  Line227 : PMComponent  Tag=PSATblock  Description=Power Flow  PhysicalDomain=psatdomain  LeftPortType=p1  RightPortType=p1  LConnTagsString=__newl0  RConnTagsString=__newr0  mask(Line){p3_4_5q=[100  115  60], p6q=10, p8q=[0.125], p9q=[0.000994719], p10q=[0.007460394e-6], p13_14_15q=[0.0 0.0 0.0], p16q=on}
      mask prompts: p3_4_5q "Power, Voltage and Frequency Ratings [MVA, kV, Hz]"; p6q "Length of line [km] (0 for p.u. parameters)"; p8q "Resistance [p.u. (Ohms/km)]"; p9q "Reactance [p.u. (H/km)]"; p10q "Susceptance [p.u. (F/km)]"; p13_14_15q "Imax, Pmax and Smax [p.u., p.u., p.u.]"; p16q "Connected"
      mask help: This block defines a pi model for a tree phase line.
      mask init:
      | [xp,yp] = fm_draw('pi');
      mask CallbackString: ||||||fm_block
      mask Display:
      | plot([-1  1  1 -1 -1],[-0.2 -0.2 0.2 0.2 -0.2])
      | color('blue')
      | plot(0.35*xp,0.2*yp)
  Line228 : PMComponent  Tag=PSATblock  Description=Power Flow  PhysicalDomain=psatdomain  LeftPortType=p1  RightPortType=p1  LConnTagsString=__newl0  RConnTagsString=__newr0  mask(Line){p3_4_5q=[100  115  60], p6q=37.45, p8q=[0.125], p9q=[0.000994719], p10q=[0.007460394e-6], p13_14_15q=[0.0 0.0 0.0], p16q=on}
      mask prompts: p3_4_5q "Power, Voltage and Frequency Ratings [MVA, kV, Hz]"; p6q "Length of line [km] (0 for p.u. parameters)"; p8q "Resistance [p.u. (Ohms/km)]"; p9q "Reactance [p.u. (H/km)]"; p10q "Susceptance [p.u. (F/km)]"; p13_14_15q "Imax, Pmax and Smax [p.u., p.u., p.u.]"; p16q "Connected"
      mask help: This block defines a pi model for a tree phase line.
      mask init:
      | [xp,yp] = fm_draw('pi');
      mask CallbackString: ||||||fm_block
      mask Display:
      | plot([-1  1  1 -1 -1],[-0.2 -0.2 0.2 0.2 -0.2])
      | color('blue')
      | plot(0.35*xp,0.2*yp)
  Line229 : PMComponent  Tag=PSATblock  Description=Power Flow  PhysicalDomain=psatdomain  LeftPortType=p1  RightPortType=p1  LConnTagsString=__newl0  RConnTagsString=__newr0  mask(Line){p3_4_5q=[100  115  60], p6q=38.92, p8q=[0.125], p9q=[0.000994719], p10q=[0.007460394e-6], p13_14_15q=[0.0 0.0 0.0], p16q=on}
      mask prompts: p3_4_5q "Power, Voltage and Frequency Ratings [MVA, kV, Hz]"; p6q "Length of line [km] (0 for p.u. parameters)"; p8q "Resistance [p.u. (Ohms/km)]"; p9q "Reactance [p.u. (H/km)]"; p10q "Susceptance [p.u. (F/km)]"; p13_14_15q "Imax, Pmax and Smax [p.u., p.u., p.u.]"; p16q "Connected"
      mask help: This block defines a pi model for a tree phase line.
      mask init:
      | [xp,yp] = fm_draw('pi');
      mask CallbackString: ||||||fm_block
      mask Display:
      | plot([-1  1  1 -1 -1],[-0.2 -0.2 0.2 0.2 -0.2])
      | color('blue')
      | plot(0.35*xp,0.2*yp)
  Line23 : PMComponent  Tag=PSATblock  Description=Power Flow  PhysicalDomain=psatdomain  LeftPortType=p1  RightPortType=p1  LConnTagsString=__newl0  RConnTagsString=__newr0  mask(Line){p3_4_5q=[100  400  60], p6q=165, p8q=[0.033806452], p9q=[0.000933966], p10q=[0.012626303e-6], p13_14_15q=[30.3 27.5 30.3], p16q=on}
      mask prompts: p3_4_5q "Power, Voltage and Frequency Ratings [MVA, kV, Hz]"; p6q "Length of line [km] (0 for p.u. parameters)"; p8q "Resistance [p.u. (Ohms/km)]"; p9q "Reactance [p.u. (H/km)]"; p10q "Susceptance [p.u. (F/km)]"; p13_14_15q "Imax, Pmax and Smax [p.u., p.u., p.u.]"; p16q "Connected"
      mask help: This block defines a pi model for a tree phase line.
      mask init:
      | [xp,yp] = fm_draw('pi');
      mask CallbackString: ||||||fm_block
      mask Display:
      | plot([-1  1  1 -1 -1],[-0.2 -0.2 0.2 0.2 -0.2])
      | color('blue')
      | plot(0.35*xp,0.2*yp)
  Line230 : PMComponent  Tag=PSATblock  Description=Power Flow  PhysicalDomain=psatdomain  LeftPortType=p1  RightPortType=p1  LConnTagsString=__newl0  RConnTagsString=__newr0  mask(Line){p3_4_5q=[100  115  60], p6q=24.14, p8q=[0.125], p9q=[0.000994719], p10q=[0.007460394e-6], p13_14_15q=[0.0 0.0 0.0], p16q=on}
      mask prompts: p3_4_5q "Power, Voltage and Frequency Ratings [MVA, kV, Hz]"; p6q "Length of line [km] (0 for p.u. parameters)"; p8q "Resistance [p.u. (Ohms/km)]"; p9q "Reactance [p.u. (H/km)]"; p10q "Susceptance [p.u. (F/km)]"; p13_14_15q "Imax, Pmax and Smax [p.u., p.u., p.u.]"; p16q "Connected"
      mask help: This block defines a pi model for a tree phase line.
      mask init:
      | [xp,yp] = fm_draw('pi');
      mask CallbackString: ||||||fm_block
      mask Display:
      | plot([-1  1  1 -1 -1],[-0.2 -0.2 0.2 0.2 -0.2])
      | color('blue')
      | plot(0.35*xp,0.2*yp)
  Line231 : PMComponent  Tag=PSATblock  Description=Power Flow  PhysicalDomain=psatdomain  LeftPortType=p1  RightPortType=p1  LConnTagsString=__newl0  RConnTagsString=__newr0  mask(Line){p3_4_5q=[100  115  60], p6q=40.38, p8q=[0.125], p9q=[0.000994719], p10q=[0.007460394e-6], p13_14_15q=[0.0 0.0 0.0], p16q=on}
      mask prompts: p3_4_5q "Power, Voltage and Frequency Ratings [MVA, kV, Hz]"; p6q "Length of line [km] (0 for p.u. parameters)"; p8q "Resistance [p.u. (Ohms/km)]"; p9q "Reactance [p.u. (H/km)]"; p10q "Susceptance [p.u. (F/km)]"; p13_14_15q "Imax, Pmax and Smax [p.u., p.u., p.u.]"; p16q "Connected"
      mask help: This block defines a pi model for a tree phase line.
      mask init:
      | [xp,yp] = fm_draw('pi');
      mask CallbackString: ||||||fm_block
      mask Display:
      | plot([-1  1  1 -1 -1],[-0.2 -0.2 0.2 0.2 -0.2])
      | color('blue')
      | plot(0.35*xp,0.2*yp)
  Line232 : PMComponent  Tag=PSATblock  Description=Power Flow  PhysicalDomain=psatdomain  LeftPortType=p1  RightPortType=p1  LConnTagsString=__newl0  RConnTagsString=__newr0  mask(Line){p3_4_5q=[100  115  60], p6q=56.35, p8q=[0.125], p9q=[0.000994719], p10q=[0.007460394e-6], p13_14_15q=[0.0 0.0 0.0], p16q=on}
      mask prompts: p3_4_5q "Power, Voltage and Frequency Ratings [MVA, kV, Hz]"; p6q "Length of line [km] (0 for p.u. parameters)"; p8q "Resistance [p.u. (Ohms/km)]"; p9q "Reactance [p.u. (H/km)]"; p10q "Susceptance [p.u. (F/km)]"; p13_14_15q "Imax, Pmax and Smax [p.u., p.u., p.u.]"; p16q "Connected"
      mask help: This block defines a pi model for a tree phase line.
      mask init:
      | [xp,yp] = fm_draw('pi');
      mask CallbackString: ||||||fm_block
      mask Display:
      | plot([-1  1  1 -1 -1],[-0.2 -0.2 0.2 0.2 -0.2])
      | color('blue')
      | plot(0.35*xp,0.2*yp)
  Line233 : PMComponent  Tag=PSATblock  Description=Power Flow  PhysicalDomain=psatdomain  LeftPortType=p1  RightPortType=p1  LConnTagsString=__newl0  RConnTagsString=__newr0  mask(Line){p3_4_5q=[100  115  60], p6q=10.81, p8q=[0.125], p9q=[0.000994719], p10q=[0.007460394e-6], p13_14_15q=[0.0 0.0 0.0], p16q=on}
      mask prompts: p3_4_5q "Power, Voltage and Frequency Ratings [MVA, kV, Hz]"; p6q "Length of line [km] (0 for p.u. parameters)"; p8q "Resistance [p.u. (Ohms/km)]"; p9q "Reactance [p.u. (H/km)]"; p10q "Susceptance [p.u. (F/km)]"; p13_14_15q "Imax, Pmax and Smax [p.u., p.u., p.u.]"; p16q "Connected"
      mask help: This block defines a pi model for a tree phase line.
      mask init:
      | [xp,yp] = fm_draw('pi');
      mask CallbackString: ||||||fm_block
      mask Display:
      | plot([-1  1  1 -1 -1],[-0.2 -0.2 0.2 0.2 -0.2])
      | color('blue')
      | plot(0.35*xp,0.2*yp)
  Line234 : PMComponent  Tag=PSATblock  Description=Power Flow  PhysicalDomain=psatdomain  LeftPortType=p1  RightPortType=p1  LConnTagsString=__newl0  RConnTagsString=__newr0  mask(Line){p3_4_5q=[100  115  60], p6q=10.81, p8q=[0.125], p9q=[0.000994719], p10q=[0.007460394e-6], p13_14_15q=[0.0 0.0 0.0], p16q=on}
      mask prompts: p3_4_5q "Power, Voltage and Frequency Ratings [MVA, kV, Hz]"; p6q "Length of line [km] (0 for p.u. parameters)"; p8q "Resistance [p.u. (Ohms/km)]"; p9q "Reactance [p.u. (H/km)]"; p10q "Susceptance [p.u. (F/km)]"; p13_14_15q "Imax, Pmax and Smax [p.u., p.u., p.u.]"; p16q "Connected"
      mask help: This block defines a pi model for a tree phase line.
      mask init:
      | [xp,yp] = fm_draw('pi');
      mask CallbackString: ||||||fm_block
      mask Display:
      | plot([-1  1  1 -1 -1],[-0.2 -0.2 0.2 0.2 -0.2])
      | color('blue')
      | plot(0.35*xp,0.2*yp)
  Line235 : PMComponent  Tag=PSATblock  Description=Power Flow  PhysicalDomain=psatdomain  LeftPortType=p1  RightPortType=p1  LConnTagsString=__newl0  RConnTagsString=__newr0  mask(Line){p3_4_5q=[100  115  60], p6q=89.17, p8q=[0.125], p9q=[0.000994719], p10q=[0.007460394e-6], p13_14_15q=[0.0 0.0 0.0], p16q=on}
      mask prompts: p3_4_5q "Power, Voltage and Frequency Ratings [MVA, kV, Hz]"; p6q "Length of line [km] (0 for p.u. parameters)"; p8q "Resistance [p.u. (Ohms/km)]"; p9q "Reactance [p.u. (H/km)]"; p10q "Susceptance [p.u. (F/km)]"; p13_14_15q "Imax, Pmax and Smax [p.u., p.u., p.u.]"; p16q "Connected"
      mask help: This block defines a pi model for a tree phase line.
      mask init:
      | [xp,yp] = fm_draw('pi');
      mask CallbackString: ||||||fm_block
      mask Display:
      | plot([-1  1  1 -1 -1],[-0.2 -0.2 0.2 0.2 -0.2])
      | color('blue')
      | plot(0.35*xp,0.2*yp)
  Line236 : PMComponent  Tag=PSATblock  Description=Power Flow  PhysicalDomain=psatdomain  LeftPortType=p1  RightPortType=p1  LConnTagsString=__newl0  RConnTagsString=__newr0  mask(Line){p3_4_5q=[100  115  60], p6q=10.71, p8q=[0.125], p9q=[0.000994719], p10q=[0.007460394e-6], p13_14_15q=[0.0 0.0 0.0], p16q=on}
      mask prompts: p3_4_5q "Power, Voltage and Frequency Ratings [MVA, kV, Hz]"; p6q "Length of line [km] (0 for p.u. parameters)"; p8q "Resistance [p.u. (Ohms/km)]"; p9q "Reactance [p.u. (H/km)]"; p10q "Susceptance [p.u. (F/km)]"; p13_14_15q "Imax, Pmax and Smax [p.u., p.u., p.u.]"; p16q "Connected"
      mask help: This block defines a pi model for a tree phase line.
      mask init:
      | [xp,yp] = fm_draw('pi');
      mask CallbackString: ||||||fm_block
      mask Display:
      | plot([-1  1  1 -1 -1],[-0.2 -0.2 0.2 0.2 -0.2])
      | color('blue')
      | plot(0.35*xp,0.2*yp)
  Line237 : PMComponent  Tag=PSATblock  Description=Power Flow  PhysicalDomain=psatdomain  LeftPortType=p1  RightPortType=p1  LConnTagsString=__newl0  RConnTagsString=__newr0  mask(Line){p3_4_5q=[100  115  60], p6q=44.90, p8q=[0.125], p9q=[0.000994719], p10q=[0.007460394e-6], p13_14_15q=[0.0 0.0 0.0], p16q=on}
      mask prompts: p3_4_5q "Power, Voltage and Frequency Ratings [MVA, kV, Hz]"; p6q "Length of line [km] (0 for p.u. parameters)"; p8q "Resistance [p.u. (Ohms/km)]"; p9q "Reactance [p.u. (H/km)]"; p10q "Susceptance [p.u. (F/km)]"; p13_14_15q "Imax, Pmax and Smax [p.u., p.u., p.u.]"; p16q "Connected"
      mask help: This block defines a pi model for a tree phase line.
      mask init:
      | [xp,yp] = fm_draw('pi');
      mask CallbackString: ||||||fm_block
      mask Display:
      | plot([-1  1  1 -1 -1],[-0.2 -0.2 0.2 0.2 -0.2])
      | color('blue')
      | plot(0.35*xp,0.2*yp)
  Line238 : PMComponent  Tag=PSATblock  Description=Power Flow  PhysicalDomain=psatdomain  LeftPortType=p1  RightPortType=p1  LConnTagsString=__newl0  RConnTagsString=__newr0  mask(Line){p3_4_5q=[100  115  60], p6q=25.69, p8q=[0.125], p9q=[0.000994719], p10q=[0.007460394e-6], p13_14_15q=[0.0 0.0 0.0], p16q=on}
      mask prompts: p3_4_5q "Power, Voltage and Frequency Ratings [MVA, kV, Hz]"; p6q "Length of line [km] (0 for p.u. parameters)"; p8q "Resistance [p.u. (Ohms/km)]"; p9q "Reactance [p.u. (H/km)]"; p10q "Susceptance [p.u. (F/km)]"; p13_14_15q "Imax, Pmax and Smax [p.u., p.u., p.u.]"; p16q "Connected"
      mask help: This block defines a pi model for a tree phase line.
      mask init:
      | [xp,yp] = fm_draw('pi');
      mask CallbackString: ||||||fm_block
      mask Display:
      | plot([-1  1  1 -1 -1],[-0.2 -0.2 0.2 0.2 -0.2])
      | color('blue')
      | plot(0.35*xp,0.2*yp)
  Line239 : PMComponent  Tag=PSATblock  Description=Power Flow  PhysicalDomain=psatdomain  LeftPortType=p1  RightPortType=p1  LConnTagsString=__newl0  RConnTagsString=__newr0  mask(Line){p3_4_5q=[100  115  60], p6q=24.55, p8q=[0.125], p9q=[0.000994719], p10q=[0.007460394e-6], p13_14_15q=[0.0 0.0 0.0], p16q=on}
      mask prompts: p3_4_5q "Power, Voltage and Frequency Ratings [MVA, kV, Hz]"; p6q "Length of line [km] (0 for p.u. parameters)"; p8q "Resistance [p.u. (Ohms/km)]"; p9q "Reactance [p.u. (H/km)]"; p10q "Susceptance [p.u. (F/km)]"; p13_14_15q "Imax, Pmax and Smax [p.u., p.u., p.u.]"; p16q "Connected"
      mask help: This block defines a pi model for a tree phase line.
      mask init:
      | [xp,yp] = fm_draw('pi');
      mask CallbackString: ||||||fm_block
      mask Display:
      | plot([-1  1  1 -1 -1],[-0.2 -0.2 0.2 0.2 -0.2])
      | color('blue')
      | plot(0.35*xp,0.2*yp)
  Line24 : PMComponent  Tag=PSATblock  Description=Power Flow  PhysicalDomain=psatdomain  LeftPortType=p1  RightPortType=p1  LConnTagsString=__newl0  RConnTagsString=__newr0  mask(Line){p3_4_5q=[100  230  60], p6q=8, p8q=[0.05], p9q=[0.001294461], p10q=[0.008941863e-6], p13_14_15q=[149 136 149], p16q=on}
      mask prompts: p3_4_5q "Power, Voltage and Frequency Ratings [MVA, kV, Hz]"; p6q "Length of line [km] (0 for p.u. parameters)"; p8q "Resistance [p.u. (Ohms/km)]"; p9q "Reactance [p.u. (H/km)]"; p10q "Susceptance [p.u. (F/km)]"; p13_14_15q "Imax, Pmax and Smax [p.u., p.u., p.u.]"; p16q "Connected"
      mask help: This block defines a pi model for a tree phase line.
      mask init:
      | [xp,yp] = fm_draw('pi');
      mask CallbackString: ||||||fm_block
      mask Display:
      | plot([-1  1  1 -1 -1],[-0.2 -0.2 0.2 0.2 -0.2])
      | color('blue')
      | plot(0.35*xp,0.2*yp)
  Line240 : PMComponent  Tag=PSATblock  Description=Power Flow  PhysicalDomain=psatdomain  LeftPortType=p1  RightPortType=p1  LConnTagsString=__newl0  RConnTagsString=__newr0  mask(Line){p3_4_5q=[100  115  60], p6q=35.97, p8q=[0.125], p9q=[0.000994719], p10q=[0.007460394e-6], p13_14_15q=[0.0 0.0 0.0], p16q=on}
      mask prompts: p3_4_5q "Power, Voltage and Frequency Ratings [MVA, kV, Hz]"; p6q "Length of line [km] (0 for p.u. parameters)"; p8q "Resistance [p.u. (Ohms/km)]"; p9q "Reactance [p.u. (H/km)]"; p10q "Susceptance [p.u. (F/km)]"; p13_14_15q "Imax, Pmax and Smax [p.u., p.u., p.u.]"; p16q "Connected"
      mask help: This block defines a pi model for a tree phase line.
      mask init:
      | [xp,yp] = fm_draw('pi');
      mask CallbackString: ||||||fm_block
      mask Display:
      | plot([-1  1  1 -1 -1],[-0.2 -0.2 0.2 0.2 -0.2])
      | color('blue')
      | plot(0.35*xp,0.2*yp)
  Line241 : PMComponent  Tag=PSATblock  Description=Power Flow  PhysicalDomain=psatdomain  LeftPortType=p1  RightPortType=p1  LConnTagsString=__newl0  RConnTagsString=__newr0  mask(Line){p3_4_5q=[100  115  60], p6q=75.21, p8q=[0.125], p9q=[0.000994719], p10q=[0.007460394e-6], p13_14_15q=[0.0 0.0 0.0], p16q=on}
      mask prompts: p3_4_5q "Power, Voltage and Frequency Ratings [MVA, kV, Hz]"; p6q "Length of line [km] (0 for p.u. parameters)"; p8q "Resistance [p.u. (Ohms/km)]"; p9q "Reactance [p.u. (H/km)]"; p10q "Susceptance [p.u. (F/km)]"; p13_14_15q "Imax, Pmax and Smax [p.u., p.u., p.u.]"; p16q "Connected"
      mask help: This block defines a pi model for a tree phase line.
      mask init:
      | [xp,yp] = fm_draw('pi');
      mask CallbackString: ||||||fm_block
      mask Display:
      | plot([-1  1  1 -1 -1],[-0.2 -0.2 0.2 0.2 -0.2])
      | color('blue')
      | plot(0.35*xp,0.2*yp)
  Line244 : PMComponent  Tag=PSATblock  Description=Power Flow  PhysicalDomain=psatdomain  LeftPortType=p1  RightPortType=p1  LConnTagsString=__newl0  RConnTagsString=__newr0  mask(Line){p3_4_5q=[100  115  60], p6q=39.24, p8q=[0.125], p9q=[0.000994719], p10q=[0.007460394e-6], p13_14_15q=[0.0 0.0 0.0], p16q=on}
      mask prompts: p3_4_5q "Power, Voltage and Frequency Ratings [MVA, kV, Hz]"; p6q "Length of line [km] (0 for p.u. parameters)"; p8q "Resistance [p.u. (Ohms/km)]"; p9q "Reactance [p.u. (H/km)]"; p10q "Susceptance [p.u. (F/km)]"; p13_14_15q "Imax, Pmax and Smax [p.u., p.u., p.u.]"; p16q "Connected"
      mask help: This block defines a pi model for a tree phase line.
      mask init:
      | [xp,yp] = fm_draw('pi');
      mask CallbackString: ||||||fm_block
      mask Display:
      | plot([-1  1  1 -1 -1],[-0.2 -0.2 0.2 0.2 -0.2])
      | color('blue')
      | plot(0.35*xp,0.2*yp)
  Line245 : PMComponent  Tag=PSATblock  Description=Power Flow  PhysicalDomain=psatdomain  LeftPortType=p1  RightPortType=p1  LConnTagsString=__newl0  RConnTagsString=__newr0  mask(Line){p3_4_5q=[100  115  60], p6q=19.52, p8q=[0.125], p9q=[0.000994719], p10q=[0.007460394e-6], p13_14_15q=[0.0 0.0 0.0], p16q=on}
      mask prompts: p3_4_5q "Power, Voltage and Frequency Ratings [MVA, kV, Hz]"; p6q "Length of line [km] (0 for p.u. parameters)"; p8q "Resistance [p.u. (Ohms/km)]"; p9q "Reactance [p.u. (H/km)]"; p10q "Susceptance [p.u. (F/km)]"; p13_14_15q "Imax, Pmax and Smax [p.u., p.u., p.u.]"; p16q "Connected"
      mask help: This block defines a pi model for a tree phase line.
      mask init:
      | [xp,yp] = fm_draw('pi');
      mask CallbackString: ||||||fm_block
      mask Display:
      | plot([-1  1  1 -1 -1],[-0.2 -0.2 0.2 0.2 -0.2])
      | color('blue')
      | plot(0.35*xp,0.2*yp)
  Line25 : PMComponent  Tag=PSATblock  Description=Power Flow  PhysicalDomain=psatdomain  LeftPortType=p1  RightPortType=p1  LConnTagsString=__newl0  RConnTagsString=__newr0  mask(Line){p3_4_5q=[100  230  60], p6q=126, p8q=[0.05], p9q=[0.001294461], p10q=[0.008941863e-6], p13_14_15q=[9.5 8.6 9.5], p16q=on}
      mask prompts: p3_4_5q "Power, Voltage and Frequency Ratings [MVA, kV, Hz]"; p6q "Length of line [km] (0 for p.u. parameters)"; p8q "Resistance [p.u. (Ohms/km)]"; p9q "Reactance [p.u. (H/km)]"; p10q "Susceptance [p.u. (F/km)]"; p13_14_15q "Imax, Pmax and Smax [p.u., p.u., p.u.]"; p16q "Connected"
      mask help: This block defines a pi model for a tree phase line.
      mask init:
      | [xp,yp] = fm_draw('pi');
      mask CallbackString: ||||||fm_block
      mask Display:
      | plot([-1  1  1 -1 -1],[-0.2 -0.2 0.2 0.2 -0.2])
      | color('blue')
      | plot(0.35*xp,0.2*yp)
  Line251 : PMComponent  Tag=PSATblock  Description=Power Flow  PhysicalDomain=psatdomain  LeftPortType=p1  RightPortType=p1  LConnTagsString=__newl0  RConnTagsString=__newr0  mask(Line){p3_4_5q=[100  115  60], p6q=39.48, p8q=[0.125], p9q=[0.000994719], p10q=[0.007460394e-6], p13_14_15q=[0.0 0.0 0.0], p16q=on}
      mask prompts: p3_4_5q "Power, Voltage and Frequency Ratings [MVA, kV, Hz]"; p6q "Length of line [km] (0 for p.u. parameters)"; p8q "Resistance [p.u. (Ohms/km)]"; p9q "Reactance [p.u. (H/km)]"; p10q "Susceptance [p.u. (F/km)]"; p13_14_15q "Imax, Pmax and Smax [p.u., p.u., p.u.]"; p16q "Connected"
      mask help: This block defines a pi model for a tree phase line.
      mask init:
      | [xp,yp] = fm_draw('pi');
      mask CallbackString: ||||||fm_block
      mask Display:
      | plot([-1  1  1 -1 -1],[-0.2 -0.2 0.2 0.2 -0.2])
      | color('blue')
      | plot(0.35*xp,0.2*yp)
  Line252 : PMComponent  Tag=PSATblock  Description=Power Flow  PhysicalDomain=psatdomain  LeftPortType=p1  RightPortType=p1  LConnTagsString=__newl0  RConnTagsString=__newr0  mask(Line){p3_4_5q=[100  115  60], p6q=28.27, p8q=[0.125], p9q=[0.000994719], p10q=[0.007460394e-6], p13_14_15q=[0.0 0.0 0.0], p16q=on}
      mask prompts: p3_4_5q "Power, Voltage and Frequency Ratings [MVA, kV, Hz]"; p6q "Length of line [km] (0 for p.u. parameters)"; p8q "Resistance [p.u. (Ohms/km)]"; p9q "Reactance [p.u. (H/km)]"; p10q "Susceptance [p.u. (F/km)]"; p13_14_15q "Imax, Pmax and Smax [p.u., p.u., p.u.]"; p16q "Connected"
      mask help: This block defines a pi model for a tree phase line.
      mask init:
      | [xp,yp] = fm_draw('pi');
      mask CallbackString: ||||||fm_block
      mask Display:
      | plot([-1  1  1 -1 -1],[-0.2 -0.2 0.2 0.2 -0.2])
      | color('blue')
      | plot(0.35*xp,0.2*yp)
  Line253 : PMComponent  Tag=PSATblock  Description=Power Flow  PhysicalDomain=psatdomain  LeftPortType=p1  RightPortType=p1  LConnTagsString=__newl0  RConnTagsString=__newr0  mask(Line){p3_4_5q=[100  115  60], p6q=51.12, p8q=[0.125], p9q=[0.000994719], p10q=[0.007460394e-6], p13_14_15q=[0.0 0.0 0.0], p16q=on}
      mask prompts: p3_4_5q "Power, Voltage and Frequency Ratings [MVA, kV, Hz]"; p6q "Length of line [km] (0 for p.u. parameters)"; p8q "Resistance [p.u. (Ohms/km)]"; p9q "Reactance [p.u. (H/km)]"; p10q "Susceptance [p.u. (F/km)]"; p13_14_15q "Imax, Pmax and Smax [p.u., p.u., p.u.]"; p16q "Connected"
      mask help: This block defines a pi model for a tree phase line.
      mask init:
      | [xp,yp] = fm_draw('pi');
      mask CallbackString: ||||||fm_block
      mask Display:
      | plot([-1  1  1 -1 -1],[-0.2 -0.2 0.2 0.2 -0.2])
      | color('blue')
      | plot(0.35*xp,0.2*yp)
  Line254 : PMComponent  Tag=PSATblock  Description=Power Flow  PhysicalDomain=psatdomain  LeftPortType=p1  RightPortType=p1  LConnTagsString=__newl0  RConnTagsString=__newr0  mask(Line){p3_4_5q=[100  115  60], p6q=52.66, p8q=[0.125], p9q=[0.000994719], p10q=[0.007460394e-6], p13_14_15q=[0.0 0.0 0.0], p16q=on}
      mask prompts: p3_4_5q "Power, Voltage and Frequency Ratings [MVA, kV, Hz]"; p6q "Length of line [km] (0 for p.u. parameters)"; p8q "Resistance [p.u. (Ohms/km)]"; p9q "Reactance [p.u. (H/km)]"; p10q "Susceptance [p.u. (F/km)]"; p13_14_15q "Imax, Pmax and Smax [p.u., p.u., p.u.]"; p16q "Connected"
      mask help: This block defines a pi model for a tree phase line.
      mask init:
      | [xp,yp] = fm_draw('pi');
      mask CallbackString: ||||||fm_block
      mask Display:
      | plot([-1  1  1 -1 -1],[-0.2 -0.2 0.2 0.2 -0.2])
      | color('blue')
      | plot(0.35*xp,0.2*yp)
  Line255 : PMComponent  Tag=PSATblock  Description=Power Flow  PhysicalDomain=psatdomain  LeftPortType=p1  RightPortType=p1  LConnTagsString=__newl0  RConnTagsString=__newr0  mask(Line){p3_4_5q=[100  115  60], p6q=52.66, p8q=[0.125], p9q=[0.000994719], p10q=[0.007460394e-6], p13_14_15q=[0.0 0.0 0.0], p16q=on}
      mask prompts: p3_4_5q "Power, Voltage and Frequency Ratings [MVA, kV, Hz]"; p6q "Length of line [km] (0 for p.u. parameters)"; p8q "Resistance [p.u. (Ohms/km)]"; p9q "Reactance [p.u. (H/km)]"; p10q "Susceptance [p.u. (F/km)]"; p13_14_15q "Imax, Pmax and Smax [p.u., p.u., p.u.]"; p16q "Connected"
      mask help: This block defines a pi model for a tree phase line.
      mask init:
      | [xp,yp] = fm_draw('pi');
      mask CallbackString: ||||||fm_block
      mask Display:
      | plot([-1  1  1 -1 -1],[-0.2 -0.2 0.2 0.2 -0.2])
      | color('blue')
      | plot(0.35*xp,0.2*yp)
  Line256 : PMComponent  Tag=PSATblock  Description=Power Flow  PhysicalDomain=psatdomain  LeftPortType=p1  RightPortType=p1  LConnTagsString=__newl0  RConnTagsString=__newr0  mask(Line){p3_4_5q=[100  115  60], p6q=41.57, p8q=[0.125], p9q=[0.000994719], p10q=[0.007460394e-6], p13_14_15q=[0.0 0.0 0.0], p16q=on}
      mask prompts: p3_4_5q "Power, Voltage and Frequency Ratings [MVA, kV, Hz]"; p6q "Length of line [km] (0 for p.u. parameters)"; p8q "Resistance [p.u. (Ohms/km)]"; p9q "Reactance [p.u. (H/km)]"; p10q "Susceptance [p.u. (F/km)]"; p13_14_15q "Imax, Pmax and Smax [p.u., p.u., p.u.]"; p16q "Connected"
      mask help: This block defines a pi model for a tree phase line.
      mask init:
      | [xp,yp] = fm_draw('pi');
      mask CallbackString: ||||||fm_block
      mask Display:
      | plot([-1  1  1 -1 -1],[-0.2 -0.2 0.2 0.2 -0.2])
      | color('blue')
      | plot(0.35*xp,0.2*yp)
  Line259 : PMComponent  Tag=PSATblock  Description=Power Flow  PhysicalDomain=psatdomain  LeftPortType=p1  RightPortType=p1  LConnTagsString=__newl0  RConnTagsString=__newr0  mask(Line){p3_4_5q=[100  115  60], p6q=34.65, p8q=[0.125], p9q=[0.000994719], p10q=[0.007460394e-6], p13_14_15q=[0.0 0.0 0.0], p16q=on}
      mask prompts: p3_4_5q "Power, Voltage and Frequency Ratings [MVA, kV, Hz]"; p6q "Length of line [km] (0 for p.u. parameters)"; p8q "Resistance [p.u. (Ohms/km)]"; p9q "Reactance [p.u. (H/km)]"; p10q "Susceptance [p.u. (F/km)]"; p13_14_15q "Imax, Pmax and Smax [p.u., p.u., p.u.]"; p16q "Connected"
      mask help: This block defines a pi model for a tree phase line.
      mask init:
      | [xp,yp] = fm_draw('pi');
      mask CallbackString: ||||||fm_block
      mask Display:
      | plot([-1  1  1 -1 -1],[-0.2 -0.2 0.2 0.2 -0.2])
      | color('blue')
      | plot(0.35*xp,0.2*yp)
  Line26 : PMComponent  Tag=PSATblock  Description=Power Flow  PhysicalDomain=psatdomain  LeftPortType=p1  RightPortType=p1  LConnTagsString=__newl0  RConnTagsString=__newr0  mask(Line){p3_4_5q=[100  230  60], p6q=20.2, p8q=[0.05], p9q=[0.001294461], p10q=[0.008941863e-6], p13_14_15q=[59 53.7 59], p16q=on}
      mask prompts: p3_4_5q "Power, Voltage and Frequency Ratings [MVA, kV, Hz]"; p6q "Length of line [km] (0 for p.u. parameters)"; p8q "Resistance [p.u. (Ohms/km)]"; p9q "Reactance [p.u. (H/km)]"; p10q "Susceptance [p.u. (F/km)]"; p13_14_15q "Imax, Pmax and Smax [p.u., p.u., p.u.]"; p16q "Connected"
      mask help: This block defines a pi model for a tree phase line.
      mask init:
      | [xp,yp] = fm_draw('pi');
      mask CallbackString: ||||||fm_block
      mask Display:
      | plot([-1  1  1 -1 -1],[-0.2 -0.2 0.2 0.2 -0.2])
      | color('blue')
      | plot(0.35*xp,0.2*yp)
  Line260 : PMComponent  Tag=PSATblock  Description=Power Flow  PhysicalDomain=psatdomain  LeftPortType=p1  RightPortType=p1  LConnTagsString=__newl0  RConnTagsString=__newr0  mask(Line){p3_4_5q=[100  115  60], p6q=56.52, p8q=[0.125], p9q=[0.000994719], p10q=[0.007460394e-6], p13_14_15q=[0.0 0.0 0.0], p16q=on}
      mask prompts: p3_4_5q "Power, Voltage and Frequency Ratings [MVA, kV, Hz]"; p6q "Length of line [km] (0 for p.u. parameters)"; p8q "Resistance [p.u. (Ohms/km)]"; p9q "Reactance [p.u. (H/km)]"; p10q "Susceptance [p.u. (F/km)]"; p13_14_15q "Imax, Pmax and Smax [p.u., p.u., p.u.]"; p16q "Connected"
      mask help: This block defines a pi model for a tree phase line.
      mask init:
      | [xp,yp] = fm_draw('pi');
      mask CallbackString: ||||||fm_block
      mask Display:
      | plot([-1  1  1 -1 -1],[-0.2 -0.2 0.2 0.2 -0.2])
      | color('blue')
      | plot(0.35*xp,0.2*yp)
  Line261 : PMComponent  Tag=PSATblock  Description=Power Flow  PhysicalDomain=psatdomain  LeftPortType=p1  RightPortType=p1  LConnTagsString=__newl0  RConnTagsString=__newr0  mask(Line){p3_4_5q=[100  115  60], p6q=62.51, p8q=[0.125], p9q=[0.000994719], p10q=[0.007460394e-6], p13_14_15q=[0.0 0.0 0.0], p16q=on}
      mask prompts: p3_4_5q "Power, Voltage and Frequency Ratings [MVA, kV, Hz]"; p6q "Length of line [km] (0 for p.u. parameters)"; p8q "Resistance [p.u. (Ohms/km)]"; p9q "Reactance [p.u. (H/km)]"; p10q "Susceptance [p.u. (F/km)]"; p13_14_15q "Imax, Pmax and Smax [p.u., p.u., p.u.]"; p16q "Connected"
      mask help: This block defines a pi model for a tree phase line.
      mask init:
      | [xp,yp] = fm_draw('pi');
      mask CallbackString: ||||||fm_block
      mask Display:
      | plot([-1  1  1 -1 -1],[-0.2 -0.2 0.2 0.2 -0.2])
      | color('blue')
      | plot(0.35*xp,0.2*yp)
  Line27 : PMComponent  Tag=PSATblock  Description=Power Flow  PhysicalDomain=psatdomain  LeftPortType=p1  RightPortType=p1  LConnTagsString=__newl0  RConnTagsString=__newr0  mask(Line){p3_4_5q=[100  400  60], p6q=210, p8q=[0.033806452], p9q=[0.000933966], p10q=[0.012626303e-6], p13_14_15q=[23.8 21.6 23.8], p16q=on}
      mask prompts: p3_4_5q "Power, Voltage and Frequency Ratings [MVA, kV, Hz]"; p6q "Length of line [km] (0 for p.u. parameters)"; p8q "Resistance [p.u. (Ohms/km)]"; p9q "Reactance [p.u. (H/km)]"; p10q "Susceptance [p.u. (F/km)]"; p13_14_15q "Imax, Pmax and Smax [p.u., p.u., p.u.]"; p16q "Connected"
      mask help: This block defines a pi model for a tree phase line.
      mask init:
      | [xp,yp] = fm_draw('pi');
      mask CallbackString: ||||||fm_block
      mask Display:
      | plot([-1  1  1 -1 -1],[-0.2 -0.2 0.2 0.2 -0.2])
      | color('blue')
      | plot(0.35*xp,0.2*yp)
  Line278 : PMComponent  Tag=PSATblock  Description=Power Flow  PhysicalDomain=psatdomain  LeftPortType=p1  RightPortType=p1  LConnTagsString=__newl0  RConnTagsString=__newr0  mask(Line){p3_4_5q=[100  115  60], p6q=14.35, p8q=[0.125], p9q=[0.000994719], p10q=[0.007460394e-6], p13_14_15q=[0.0 0.0 0.0], p16q=on}
      mask prompts: p3_4_5q "Power, Voltage and Frequency Ratings [MVA, kV, Hz]"; p6q "Length of line [km] (0 for p.u. parameters)"; p8q "Resistance [p.u. (Ohms/km)]"; p9q "Reactance [p.u. (H/km)]"; p10q "Susceptance [p.u. (F/km)]"; p13_14_15q "Imax, Pmax and Smax [p.u., p.u., p.u.]"; p16q "Connected"
      mask help: This block defines a pi model for a tree phase line.
      mask init:
      | [xp,yp] = fm_draw('pi');
      mask CallbackString: ||||||fm_block
      mask Display:
      | plot([-1  1  1 -1 -1],[-0.2 -0.2 0.2 0.2 -0.2])
      | color('blue')
      | plot(0.35*xp,0.2*yp)
  Line279 : PMComponent  Tag=PSATblock  Description=Power Flow  PhysicalDomain=psatdomain  LeftPortType=p1  RightPortType=p1  LConnTagsString=__newl0  RConnTagsString=__newr0  mask(Line){p3_4_5q=[100  115  60], p6q=12.81, p8q=[0.125], p9q=[0.000994719], p10q=[0.007460394e-6], p13_14_15q=[0.0 0.0 0.0], p16q=on}
      mask prompts: p3_4_5q "Power, Voltage and Frequency Ratings [MVA, kV, Hz]"; p6q "Length of line [km] (0 for p.u. parameters)"; p8q "Resistance [p.u. (Ohms/km)]"; p9q "Reactance [p.u. (H/km)]"; p10q "Susceptance [p.u. (F/km)]"; p13_14_15q "Imax, Pmax and Smax [p.u., p.u., p.u.]"; p16q "Connected"
      mask help: This block defines a pi model for a tree phase line.
      mask init:
      | [xp,yp] = fm_draw('pi');
      mask CallbackString: ||||||fm_block
      mask Display:
      | plot([-1  1  1 -1 -1],[-0.2 -0.2 0.2 0.2 -0.2])
      | color('blue')
      | plot(0.35*xp,0.2*yp)
  Line28 : PMComponent  Tag=PSATblock  Description=Power Flow  PhysicalDomain=psatdomain  LeftPortType=p1  RightPortType=p1  LConnTagsString=__newl0  RConnTagsString=__newr0  mask(Line){p3_4_5q=[100  230  60], p6q=142, p8q=[0.05], p9q=[0.001294461], p10q=[0.008941863e-6], p13_14_15q=[8.4 7.6 8.4], p16q=on}
      mask prompts: p3_4_5q "Power, Voltage and Frequency Ratings [MVA, kV, Hz]"; p6q "Length of line [km] (0 for p.u. parameters)"; p8q "Resistance [p.u. (Ohms/km)]"; p9q "Reactance [p.u. (H/km)]"; p10q "Susceptance [p.u. (F/km)]"; p13_14_15q "Imax, Pmax and Smax [p.u., p.u., p.u.]"; p16q "Connected"
      mask help: This block defines a pi model for a tree phase line.
      mask init:
      | [xp,yp] = fm_draw('pi');
      mask CallbackString: ||||||fm_block
      mask Display:
      | plot([-1  1  1 -1 -1],[-0.2 -0.2 0.2 0.2 -0.2])
      | color('blue')
      | plot(0.35*xp,0.2*yp)
  Line280 : PMComponent  Tag=PSATblock  Description=Power Flow  PhysicalDomain=psatdomain  LeftPortType=p1  RightPortType=p1  LConnTagsString=__newl0  RConnTagsString=__newr0  mask(Line){p3_4_5q=[100  115  60], p6q=12.81, p8q=[0.125], p9q=[0.000994719], p10q=[0.007460394e-6], p13_14_15q=[0.0 0.0 0.0], p16q=on}
      mask prompts: p3_4_5q "Power, Voltage and Frequency Ratings [MVA, kV, Hz]"; p6q "Length of line [km] (0 for p.u. parameters)"; p8q "Resistance [p.u. (Ohms/km)]"; p9q "Reactance [p.u. (H/km)]"; p10q "Susceptance [p.u. (F/km)]"; p13_14_15q "Imax, Pmax and Smax [p.u., p.u., p.u.]"; p16q "Connected"
      mask help: This block defines a pi model for a tree phase line.
      mask init:
      | [xp,yp] = fm_draw('pi');
      mask CallbackString: ||||||fm_block
      mask Display:
      | plot([-1  1  1 -1 -1],[-0.2 -0.2 0.2 0.2 -0.2])
      | color('blue')
      | plot(0.35*xp,0.2*yp)
  Line281 : PMComponent  Tag=PSATblock  Description=Power Flow  PhysicalDomain=psatdomain  LeftPortType=p1  RightPortType=p1  LConnTagsString=__newl0  RConnTagsString=__newr0  mask(Line){p3_4_5q=[100  115  60], p6q=10, p8q=[0.125], p9q=[0.000994719], p10q=[0.007460394e-6], p13_14_15q=[0.0 0.0 0.0], p16q=on}
      mask prompts: p3_4_5q "Power, Voltage and Frequency Ratings [MVA, kV, Hz]"; p6q "Length of line [km] (0 for p.u. parameters)"; p8q "Resistance [p.u. (Ohms/km)]"; p9q "Reactance [p.u. (H/km)]"; p10q "Susceptance [p.u. (F/km)]"; p13_14_15q "Imax, Pmax and Smax [p.u., p.u., p.u.]"; p16q "Connected"
      mask help: This block defines a pi model for a tree phase line.
      mask init:
      | [xp,yp] = fm_draw('pi');
      mask CallbackString: ||||||fm_block
      mask Display:
      | plot([-1  1  1 -1 -1],[-0.2 -0.2 0.2 0.2 -0.2])
      | color('blue')
      | plot(0.35*xp,0.2*yp)
  Line282 : PMComponent  Tag=PSATblock  Description=Power Flow  PhysicalDomain=psatdomain  LeftPortType=p1  RightPortType=p1  LConnTagsString=__newl0  RConnTagsString=__newr0  mask(Line){p3_4_5q=[100  115  60], p6q=7.55, p8q=[0.125], p9q=[0.000994719], p10q=[0.007460394e-6], p13_14_15q=[0.0 0.0 0.0], p16q=on}
      mask prompts: p3_4_5q "Power, Voltage and Frequency Ratings [MVA, kV, Hz]"; p6q "Length of line [km] (0 for p.u. parameters)"; p8q "Resistance [p.u. (Ohms/km)]"; p9q "Reactance [p.u. (H/km)]"; p10q "Susceptance [p.u. (F/km)]"; p13_14_15q "Imax, Pmax and Smax [p.u., p.u., p.u.]"; p16q "Connected"
      mask help: This block defines a pi model for a tree phase line.
      mask init:
      | [xp,yp] = fm_draw('pi');
      mask CallbackString: ||||||fm_block
      mask Display:
      | plot([-1  1  1 -1 -1],[-0.2 -0.2 0.2 0.2 -0.2])
      | color('blue')
      | plot(0.35*xp,0.2*yp)
  Line283 : PMComponent  Tag=PSATblock  Description=Power Flow  PhysicalDomain=psatdomain  LeftPortType=p1  RightPortType=p1  LConnTagsString=__newl0  RConnTagsString=__newr0  mask(Line){p3_4_5q=[100  115  60], p6q=35.54, p8q=[0.125], p9q=[0.000994719], p10q=[0.007460394e-6], p13_14_15q=[0.0 0.0 0.0], p16q=on}
      mask prompts: p3_4_5q "Power, Voltage and Frequency Ratings [MVA, kV, Hz]"; p6q "Length of line [km] (0 for p.u. parameters)"; p8q "Resistance [p.u. (Ohms/km)]"; p9q "Reactance [p.u. (H/km)]"; p10q "Susceptance [p.u. (F/km)]"; p13_14_15q "Imax, Pmax and Smax [p.u., p.u., p.u.]"; p16q "Connected"
      mask help: This block defines a pi model for a tree phase line.
      mask init:
      | [xp,yp] = fm_draw('pi');
      mask CallbackString: ||||||fm_block
      mask Display:
      | plot([-1  1  1 -1 -1],[-0.2 -0.2 0.2 0.2 -0.2])
      | color('blue')
      | plot(0.35*xp,0.2*yp)
  Line29 : PMComponent  Tag=PSATblock  Description=Power Flow  PhysicalDomain=psatdomain  LeftPortType=p1  RightPortType=p1  LConnTagsString=__newl0  RConnTagsString=__newr0  mask(Line){p3_4_5q=[100  230  60], p6q=21, p8q=[0.05], p9q=[0.001294461], p10q=[0.008941863e-6], p13_14_15q=[56.8 51.5 56.8], p16q=on}
      mask prompts: p3_4_5q "Power, Voltage and Frequency Ratings [MVA, kV, Hz]"; p6q "Length of line [km] (0 for p.u. parameters)"; p8q "Resistance [p.u. (Ohms/km)]"; p9q "Reactance [p.u. (H/km)]"; p10q "Susceptance [p.u. (F/km)]"; p13_14_15q "Imax, Pmax and Smax [p.u., p.u., p.u.]"; p16q "Connected"
      mask help: This block defines a pi model for a tree phase line.
      mask init:
      | [xp,yp] = fm_draw('pi');
      mask CallbackString: ||||||fm_block
      mask Display:
      | plot([-1  1  1 -1 -1],[-0.2 -0.2 0.2 0.2 -0.2])
      | color('blue')
      | plot(0.35*xp,0.2*yp)
  Line3 : PMComponent  Tag=PSATblock  Description=Power Flow  PhysicalDomain=psatdomain  LeftPortType=p1  RightPortType=p1  LConnTagsString=__newl0  RConnTagsString=__newr0  mask(Line){p3_4_5q=[100  765  60], p6q=[225], p8q=[0.012], p9q=[0.0008727], p10q=[0.013204566e-6], p13_14_15q=[25.29 22.76 25.29], p16q=on}
      mask prompts: p3_4_5q "Power, Voltage and Frequency Ratings [MVA, kV, Hz]"; p6q "Length of line [km] (0 for p.u. parameters)"; p8q "Resistance [p.u. (Ohms/km)]"; p9q "Reactance [p.u. (H/km)]"; p10q "Susceptance [p.u. (F/km)]"; p13_14_15q "Imax, Pmax and Smax [p.u., p.u., p.u.]"; p16q "Connected"
      mask help: This block defines a pi model for a tree phase line.
      mask init:
      | [xp,yp] = fm_draw('pi');
      mask CallbackString: ||||||fm_block
      mask Display:
      | plot([-1  1  1 -1 -1],[-0.2 -0.2 0.2 0.2 -0.2])
      | color('blue')
      | plot(0.35*xp,0.2*yp)
  Line30 : PMComponent  Tag=PSATblock  Description=Power Flow  PhysicalDomain=psatdomain  LeftPortType=p1  RightPortType=p1  LConnTagsString=__newl0  RConnTagsString=__newr0  mask(Line){p3_4_5q=[100  230  60], p6q=31, p8q=[0.05], p9q=[0.001294461], p10q=[0.008941863e-6], p13_14_15q=[38.5 35 38.5], p16q=on}
      mask prompts: p3_4_5q "Power, Voltage and Frequency Ratings [MVA, kV, Hz]"; p6q "Length of line [km] (0 for p.u. parameters)"; p8q "Resistance [p.u. (Ohms/km)]"; p9q "Reactance [p.u. (H/km)]"; p10q "Susceptance [p.u. (F/km)]"; p13_14_15q "Imax, Pmax and Smax [p.u., p.u., p.u.]"; p16q "Connected"
      mask help: This block defines a pi model for a tree phase line.
      mask init:
      | [xp,yp] = fm_draw('pi');
      mask CallbackString: ||||||fm_block
      mask Display:
      | plot([-1  1  1 -1 -1],[-0.2 -0.2 0.2 0.2 -0.2])
      | color('blue')
      | plot(0.35*xp,0.2*yp)
  Line31 : PMComponent  Tag=PSATblock  Description=Power Flow  PhysicalDomain=psatdomain  LeftPortType=p1  RightPortType=p1  LConnTagsString=__newl0  RConnTagsString=__newr0  mask(Line){p3_4_5q=[100  230  60], p6q=142, p8q=[0.05], p9q=[0.001294461], p10q=[0.008941863e-6], p13_14_15q=[8.4 7.6 8.4], p16q=on}
      mask prompts: p3_4_5q "Power, Voltage and Frequency Ratings [MVA, kV, Hz]"; p6q "Length of line [km] (0 for p.u. parameters)"; p8q "Resistance [p.u. (Ohms/km)]"; p9q "Reactance [p.u. (H/km)]"; p10q "Susceptance [p.u. (F/km)]"; p13_14_15q "Imax, Pmax and Smax [p.u., p.u., p.u.]"; p16q "Connected"
      mask help: This block defines a pi model for a tree phase line.
      mask init:
      | [xp,yp] = fm_draw('pi');
      mask CallbackString: ||||||fm_block
      mask Display:
      | plot([-1  1  1 -1 -1],[-0.2 -0.2 0.2 0.2 -0.2])
      | color('blue')
      | plot(0.35*xp,0.2*yp)
  Line32 : PMComponent  Tag=PSATblock  Description=Power Flow  PhysicalDomain=psatdomain  LeftPortType=p1  RightPortType=p1  LConnTagsString=__newl0  RConnTagsString=__newr0  mask(Line){p3_4_5q=[100  230  60], p6q=100, p8q=[0.05], p9q=[0.001294461], p10q=[0.008941863e-6], p13_14_15q=[11.9 10.8 11.9], p16q=on}
      mask prompts: p3_4_5q "Power, Voltage and Frequency Ratings [MVA, kV, Hz]"; p6q "Length of line [km] (0 for p.u. parameters)"; p8q "Resistance [p.u. (Ohms/km)]"; p9q "Reactance [p.u. (H/km)]"; p10q "Susceptance [p.u. (F/km)]"; p13_14_15q "Imax, Pmax and Smax [p.u., p.u., p.u.]"; p16q "Connected"
      mask help: This block defines a pi model for a tree phase line.
      mask init:
      | [xp,yp] = fm_draw('pi');
      mask CallbackString: ||||||fm_block
      mask Display:
      | plot([-1  1  1 -1 -1],[-0.2 -0.2 0.2 0.2 -0.2])
      | color('blue')
      | plot(0.35*xp,0.2*yp)
  Line33 : PMComponent  Tag=PSATblock  Description=Power Flow  PhysicalDomain=psatdomain  LeftPortType=p1  RightPortType=p1  LConnTagsString=__newl0  RConnTagsString=__newr0  mask(Line){p3_4_5q=[100  230  60], p6q=64, p8q=[0.05], p9q=[0.001294461], p10q=[0.008941863e-6], p13_14_15q=[18.6 16.9 18.6], p16q=on}
      mask prompts: p3_4_5q "Power, Voltage and Frequency Ratings [MVA, kV, Hz]"; p6q "Length of line [km] (0 for p.u. parameters)"; p8q "Resistance [p.u. (Ohms/km)]"; p9q "Reactance [p.u. (H/km)]"; p10q "Susceptance [p.u. (F/km)]"; p13_14_15q "Imax, Pmax and Smax [p.u., p.u., p.u.]"; p16q "Connected"
      mask help: This block defines a pi model for a tree phase line.
      mask init:
      | [xp,yp] = fm_draw('pi');
      mask CallbackString: ||||||fm_block
      mask Display:
      | plot([-1  1  1 -1 -1],[-0.2 -0.2 0.2 0.2 -0.2])
      | color('blue')
      | plot(0.35*xp,0.2*yp)
  Line34 : PMComponent  Tag=PSATblock  Description=Power Flow  PhysicalDomain=psatdomain  LeftPortType=p1  RightPortType=p1  LConnTagsString=__newl0  RConnTagsString=__newr0  mask(Line){p3_4_5q=[100  230  60], p6q=148, p8q=[0.05], p9q=[0.001294461], p10q=[0.008941863e-6], p13_14_15q=[8.1 7.3 8.1], p16q=on}
      mask prompts: p3_4_5q "Power, Voltage and Frequency Ratings [MVA, kV, Hz]"; p6q "Length of line [km] (0 for p.u. parameters)"; p8q "Resistance [p.u. (Ohms/km)]"; p9q "Reactance [p.u. (H/km)]"; p10q "Susceptance [p.u. (F/km)]"; p13_14_15q "Imax, Pmax and Smax [p.u., p.u., p.u.]"; p16q "Connected"
      mask help: This block defines a pi model for a tree phase line.
      mask init:
      | [xp,yp] = fm_draw('pi');
      mask CallbackString: ||||||fm_block
      mask Display:
      | plot([-1  1  1 -1 -1],[-0.2 -0.2 0.2 0.2 -0.2])
      | color('blue')
      | plot(0.35*xp,0.2*yp)
  Line35 : PMComponent  Tag=PSATblock  Description=Power Flow  PhysicalDomain=psatdomain  LeftPortType=p1  RightPortType=p1  LConnTagsString=__newl0  RConnTagsString=__newr0  mask(Line){p3_4_5q=[100  400  60], p6q=164, p8q=[0.033806452], p9q=[0.000933966], p10q=[0.012626303e-6], p13_14_15q=[30.5 27.7 30.5], p16q=on}
      mask prompts: p3_4_5q "Power, Voltage and Frequency Ratings [MVA, kV, Hz]"; p6q "Length of line [km] (0 for p.u. parameters)"; p8q "Resistance [p.u. (Ohms/km)]"; p9q "Reactance [p.u. (H/km)]"; p10q "Susceptance [p.u. (F/km)]"; p13_14_15q "Imax, Pmax and Smax [p.u., p.u., p.u.]"; p16q "Connected"
      mask help: This block defines a pi model for a tree phase line.
      mask init:
      | [xp,yp] = fm_draw('pi');
      mask CallbackString: ||||||fm_block
      mask Display:
      | plot([-1  1  1 -1 -1],[-0.2 -0.2 0.2 0.2 -0.2])
      | color('blue')
      | plot(0.35*xp,0.2*yp)
  Line36 : PMComponent  Tag=PSATblock  Description=Power Flow  PhysicalDomain=psatdomain  LeftPortType=p1  RightPortType=p1  LConnTagsString=__newl0  RConnTagsString=__newr0  mask(Line){p3_4_5q=[100  230  60], p6q=126, p8q=[0.05], p9q=[0.001294461], p10q=[0.008941863e-6], p13_14_15q=[9.5 8.6 9.5], p16q=on}
      mask prompts: p3_4_5q "Power, Voltage and Frequency Ratings [MVA, kV, Hz]"; p6q "Length of line [km] (0 for p.u. parameters)"; p8q "Resistance [p.u. (Ohms/km)]"; p9q "Reactance [p.u. (H/km)]"; p10q "Susceptance [p.u. (F/km)]"; p13_14_15q "Imax, Pmax and Smax [p.u., p.u., p.u.]"; p16q "Connected"
      mask help: This block defines a pi model for a tree phase line.
      mask init:
      | [xp,yp] = fm_draw('pi');
      mask CallbackString: ||||||fm_block
      mask Display:
      | plot([-1  1  1 -1 -1],[-0.2 -0.2 0.2 0.2 -0.2])
      | color('blue')
      | plot(0.35*xp,0.2*yp)
  Line37 : PMComponent  Tag=PSATblock  Description=Power Flow  PhysicalDomain=psatdomain  LeftPortType=p1  RightPortType=p1  LConnTagsString=__newl0  RConnTagsString=__newr0  mask(Line){p3_4_5q=[100  230  60], p6q=192, p8q=[0.05], p9q=[0.001294461], p10q=[0.008941863e-6], p13_14_15q=[6.2 5.6 6.2], p16q=on}
      mask prompts: p3_4_5q "Power, Voltage and Frequency Ratings [MVA, kV, Hz]"; p6q "Length of line [km] (0 for p.u. parameters)"; p8q "Resistance [p.u. (Ohms/km)]"; p9q "Reactance [p.u. (H/km)]"; p10q "Susceptance [p.u. (F/km)]"; p13_14_15q "Imax, Pmax and Smax [p.u., p.u., p.u.]"; p16q "Connected"
      mask help: This block defines a pi model for a tree phase line.
      mask init:
      | [xp,yp] = fm_draw('pi');
      mask CallbackString: ||||||fm_block
      mask Display:
      | plot([-1  1  1 -1 -1],[-0.2 -0.2 0.2 0.2 -0.2])
      | color('blue')
      | plot(0.35*xp,0.2*yp)
  Line38 : PMComponent  Tag=PSATblock  Description=Power Flow  PhysicalDomain=psatdomain  LeftPortType=p1  RightPortType=p1  LConnTagsString=__newl0  RConnTagsString=__newr0  mask(Line){p3_4_5q=[100  400  60], p6q=10, p8q=[0.033806452], p9q=[0.000933966], p10q=[0.012626303e-6], p13_14_15q=[500 454 500], p16q=on}
      mask prompts: p3_4_5q "Power, Voltage and Frequency Ratings [MVA, kV, Hz]"; p6q "Length of line [km] (0 for p.u. parameters)"; p8q "Resistance [p.u. (Ohms/km)]"; p9q "Reactance [p.u. (H/km)]"; p10q "Susceptance [p.u. (F/km)]"; p13_14_15q "Imax, Pmax and Smax [p.u., p.u., p.u.]"; p16q "Connected"
      mask help: This block defines a pi model for a tree phase line.
      mask init:
      | [xp,yp] = fm_draw('pi');
      mask CallbackString: ||||||fm_block
      mask Display:
      | plot([-1  1  1 -1 -1],[-0.2 -0.2 0.2 0.2 -0.2])
      | color('blue')
      | plot(0.35*xp,0.2*yp)
  Line39 : PMComponent  Tag=PSATblock  Description=Power Flow  PhysicalDomain=psatdomain  LeftPortType=p1  RightPortType=p1  LConnTagsString=__newl0  RConnTagsString=__newr0  mask(Line){p3_4_5q=[100  765  60], p6q=[182], p8q=[0.012], p9q=[0.0008727], p10q=[0.013204566e-6], p13_14_15q=[25.29 22.76 25.29], p16q=on}
      mask prompts: p3_4_5q "Power, Voltage and Frequency Ratings [MVA, kV, Hz]"; p6q "Length of line [km] (0 for p.u. parameters)"; p8q "Resistance [p.u. (Ohms/km)]"; p9q "Reactance [p.u. (H/km)]"; p10q "Susceptance [p.u. (F/km)]"; p13_14_15q "Imax, Pmax and Smax [p.u., p.u., p.u.]"; p16q "Connected"
      mask help: This block defines a pi model for a tree phase line.
      mask init:
      | [xp,yp] = fm_draw('pi');
      mask CallbackString: ||||||fm_block
      mask Display:
      | plot([-1  1  1 -1 -1],[-0.2 -0.2 0.2 0.2 -0.2])
      | color('blue')
      | plot(0.35*xp,0.2*yp)
  Line4 : PMComponent  Tag=PSATblock  Description=Power Flow  PhysicalDomain=psatdomain  LeftPortType=p1  RightPortType=p1  LConnTagsString=__newl0  RConnTagsString=__newr0  mask(Line){p3_4_5q=[100  765  60], p6q=[225], p8q=[0.012], p9q=[0.0008727], p10q=[0.013204566e-6], p13_14_15q=[25.29 22.76 25.29], p16q=on}
      mask prompts: p3_4_5q "Power, Voltage and Frequency Ratings [MVA, kV, Hz]"; p6q "Length of line [km] (0 for p.u. parameters)"; p8q "Resistance [p.u. (Ohms/km)]"; p9q "Reactance [p.u. (H/km)]"; p10q "Susceptance [p.u. (F/km)]"; p13_14_15q "Imax, Pmax and Smax [p.u., p.u., p.u.]"; p16q "Connected"
      mask help: This block defines a pi model for a tree phase line.
      mask init:
      | [xp,yp] = fm_draw('pi');
      mask CallbackString: ||||||fm_block
      mask Display:
      | plot([-1  1  1 -1 -1],[-0.2 -0.2 0.2 0.2 -0.2])
      | color('blue')
      | plot(0.35*xp,0.2*yp)
  Line40 : PMComponent  Tag=PSATblock  Description=Power Flow  PhysicalDomain=psatdomain  LeftPortType=p1  RightPortType=p1  LConnTagsString=__newl0  RConnTagsString=__newr0  mask(Line){p3_4_5q=[100  765  60], p6q=[90], p8q=[0.012], p9q=[0.0008727], p10q=[0.013204566e-6], p13_14_15q=[25.29 22.76 25.29], p16q=on}
      mask prompts: p3_4_5q "Power, Voltage and Frequency Ratings [MVA, kV, Hz]"; p6q "Length of line [km] (0 for p.u. parameters)"; p8q "Resistance [p.u. (Ohms/km)]"; p9q "Reactance [p.u. (H/km)]"; p10q "Susceptance [p.u. (F/km)]"; p13_14_15q "Imax, Pmax and Smax [p.u., p.u., p.u.]"; p16q "Connected"
      mask help: This block defines a pi model for a tree phase line.
      mask init:
      | [xp,yp] = fm_draw('pi');
      mask CallbackString: ||||||fm_block
      mask Display:
      | plot([-1  1  1 -1 -1],[-0.2 -0.2 0.2 0.2 -0.2])
      | color('blue')
      | plot(0.35*xp,0.2*yp)
  Line41 : PMComponent  Tag=PSATblock  Description=Power Flow  PhysicalDomain=psatdomain  LeftPortType=p1  RightPortType=p1  LConnTagsString=__newl0  RConnTagsString=__newr0  mask(Line){p3_4_5q=[100,765,60], p6q=123, p8q=[0.012], p9q=[0.0008727], p10q=[0.013204566e-6], p13_14_15q=[25.29 22.76 25.29], p16q=on}
      mask prompts: p3_4_5q "Power, Voltage and Frequency Ratings [MVA, kV, Hz]"; p6q "Length of line [km] (0 for p.u. parameters)"; p8q "Resistance [p.u. (Ohms/km)]"; p9q "Reactance [p.u. (H/km)]"; p10q "Susceptance [p.u. (F/km)]"; p13_14_15q "Imax, Pmax and Smax [p.u., p.u., p.u.]"; p16q "Connected"
      mask help: This block defines a pi model for a tree phase line.
      mask init:
      | [xp,yp] = fm_draw('pi');
      mask CallbackString: ||||||fm_block
      mask Display:
      | plot([-1  1  1 -1 -1],[-0.2 -0.2 0.2 0.2 -0.2])
      | color('blue')
      | plot(0.35*xp,0.2*yp)
  Line42 : PMComponent  Tag=PSATblock  Description=Power Flow  PhysicalDomain=psatdomain  LeftPortType=p1  RightPortType=p1  LConnTagsString=__newl0  RConnTagsString=__newr0  mask(Line){p3_4_5q=[100,765,60], p6q=123, p8q=[0.012], p9q=[0.0008727], p10q=[0.013204566e-6], p13_14_15q=[25.29 22.76 25.29], p16q=on}
      mask prompts: p3_4_5q "Power, Voltage and Frequency Ratings [MVA, kV, Hz]"; p6q "Length of line [km] (0 for p.u. parameters)"; p8q "Resistance [p.u. (Ohms/km)]"; p9q "Reactance [p.u. (H/km)]"; p10q "Susceptance [p.u. (F/km)]"; p13_14_15q "Imax, Pmax and Smax [p.u., p.u., p.u.]"; p16q "Connected"
      mask help: This block defines a pi model for a tree phase line.
      mask init:
      | [xp,yp] = fm_draw('pi');
      mask CallbackString: ||||||fm_block
      mask Display:
      | plot([-1  1  1 -1 -1],[-0.2 -0.2 0.2 0.2 -0.2])
      | color('blue')
      | plot(0.35*xp,0.2*yp)
  Line43 : PMComponent  Tag=PSATblock  Description=Power Flow  PhysicalDomain=psatdomain  LeftPortType=p1  RightPortType=p1  LConnTagsString=__newl0  RConnTagsString=__newr0  mask(Line){p3_4_5q=[100  765  60], p6q=[270], p8q=[0.012], p9q=[0.0008727], p10q=[0.013204566e-6], p13_14_15q=[25.29 22.76 25.29], p16q=on}
